simulink model "ssc_Probes_test_all"  (R2019b)
settings: Solver=ode23t  StartTime=0.0  StopTime=10.0  RelTol=1e-3  EnableMultiTasking=on
undefined symbols (not defined in the file): damping_coeff
libraries: fl_lib x88, nesl_utility x71, Pneumatic_lib x16, fl_ps_legacy_lib x1
(part 1 of 4)
settings Model: Creator=tegel  LastModifiedBy=bhisma
settings DataIOCC: LimitDataPoints=on  SaveFormat=Array  ReturnWorkspaceOutputs=off
settings OptimizationCC: ExpressionDepthLimit=2147483647  LifeSpan=inf
settings DebuggingCC: UnderspecifiedInitializationDetection=Classic  MergeDetectMultiDrivingBlocksExec=none  SolverPrmCheckMsg=warning  StateNameClashWarn=warning  SFUnexpectedBacktrackingDiag=warning  SFNoUnconditionalDefaultTransitionDiag=warning  SFExecutionAtInitializationDiag=none  ArithmeticOperatorsInVariantConditions=warning
settings HardwareCC: ProdBitPerPointer=32  ProdBitPerSizeT=32  ProdBitPerPtrDiffT=32  ProdLargestAtomicFloat=None  ProdIntDivRoundTo=Undefined  ProdEndianess=Unspecified  ProdWordSize=32  ProdHWDeviceType=32-bit Generic
settings ModelReferenceCC: PropagateSignalLabelsOutOfModel=off
settings SFSimCC: SimUseLocalCustomCode=off  CustomCodeUndefinedFunction=UseInterfaceOnly
settings RTWCC: RTWUseLocalCustomCode=off
settings CodeAppCC: StateflowObjectComments=on
settings GRTTargetCC: TargetLangStandard=C89/C90 (ANSI)  GeneratePreprocessorConditionals=Disable all
settings ConfigComp: CovMetricSettings=dw  CovHtmlReporting=on  CovSaveCumulativeToWorkspaceVar=on  CovSaveSingleToWorkspaceVar=on  CovExternalEMLEnable=off  CovSFcnEnable=off
settings SimscapeCC: SimscapeNormalizeSystem=off

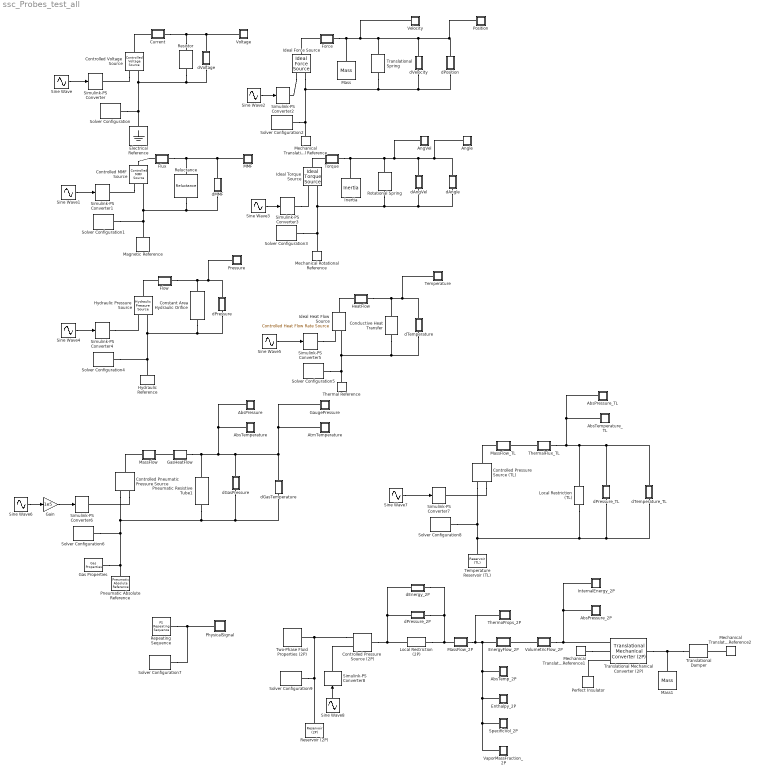
== system ssc_Probes_test_all ==
  AbsPressure : Subsystem  Description=Simscape Probe  InitFcn=|
      | unit=get_param([gcb '/PS-S'],'Unit');                                              
      | set_param(gcb, 'AttributesFormatString', strcat('[', unit,']'));
      mask help: Simscape Probe
      settings: AttributesFormatString=[Pa]
      settings: CopyFcn=|
      | set_param(gcb,'LinkStatus','inactive');
      | set_param(gcb,'LinkStatus','none');
      | set_param([gcb '/Goto'],'GotoTag', [get(gcbh,'name')]);
      | set_param([gcb '/From'],'GotoTag', [get(gcbh,'name')]);
      | h = get_param([gcb, '/PS-S'], 'PortHandles');
      | set(h.Outport(1), 'SignalNameFromLabel', [get(gcbh,'name')])
      | clear h;
      settings: NameChangeFcn=|
      | set_param([gcb '/Goto'],'GotoTag', [get(gcbh,'name')]);
      | set_param([gcb '/From'],'GotoTag', [get(gcbh,'name')]);
      | h = get_param([gcb, '/PS-S'], 'PortHandles');
      | set(h.Outport(1), 'SignalNameFromLabel', [get(gcbh,'name')])
      | clear h;
      settings: OpenFcn=|
      | if exist('logsout', 'var')
      |   vname = get(gcbh,'name');
      |   fHandle = findall(0,'Tag',vname);
      |   if isempty(fHandle)
      |   figure('Tag',vname);
      |   end;
      |   figure(findobj('Tag',vname));
      |   plot(logsout.getElement([gcb, '/PS-S'], '-blockpath').Values)
      |   title(get(gcbh,'name'));
      |   ylabel(['Pressure (' get_param([gcb '/PS-S'],'Unit') ')'] );
      | end
      mask Display: port_label('LConn', 1,'P');
  AbsPressure_2P : Subsystem  Description=Simscape Probe  InitFcn=|
      | unit=get_param([gcb '/PS-S'],'Unit');                                              
      | set_param(gcb, 'AttributesFormatString', strcat('[', unit,']'));
      mask help: Simscape Probe
      settings: AttributesFormatString=[Pa]
      settings: CopyFcn=|
      | set_param(gcb,'LinkStatus','inactive');
      | set_param(gcb,'LinkStatus','none');
      | set_param([gcb '/Goto'],'GotoTag', [get(gcbh,'name')]);
      | set_param([gcb '/From'],'GotoTag', [get(gcbh,'name')]);
      | h = get_param([gcb, '/PS-S'], 'PortHandles');
      | set(h.Outport(1), 'SignalNameFromLabel', [get(gcbh,'name')])
      | clear h;
      settings: NameChangeFcn=|
      | set_param([gcb '/Goto'],'GotoTag', [get(gcbh,'name')]);
      | set_param([gcb '/From'],'GotoTag', [get(gcbh,'name')]);
      | h = get_param([gcb, '/PS-S'], 'PortHandles');
      | set(h.Outport(1), 'SignalNameFromLabel', [get(gcbh,'name')])
      | clear h;
      settings: OpenFcn=|
      | if exist('logsout', 'var')
      |   vname = get(gcbh,'name');
      |   fHandle = findall(0,'Tag',vname);
      |   if isempty(fHandle)
      |   figure('Tag',vname);
      |   end;
      |   figure(findobj('Tag',vname));
      |   plot(logsout.getElement([gcb, '/PS-S'], '-blockpath').Values)
      |   title(get(gcbh,'name'));
      |   ylabel(['Pressure (' get_param([gcb '/PS-S'],'Unit') ')'] );
      | end
      mask Display: port_label('LConn', 1,'P');
  AbsPressure_TL : Subsystem  Description=Simscape Probe  InitFcn=|
      | unit=get_param([gcb '/PS-S'],'Unit');                                              
      | set_param(gcb, 'AttributesFormatString', strcat('[', unit,']'));
      mask help: Simscape Probe
      settings: AttributesFormatString=[Pa]
      settings: CopyFcn=|
      | set_param(gcb,'LinkStatus','inactive');
      | set_param(gcb,'LinkStatus','none');
      | set_param([gcb '/Goto'],'GotoTag', [get(gcbh,'name')]);
      | set_param([gcb '/From'],'GotoTag', [get(gcbh,'name')]);
      | h = get_param([gcb, '/PS-S'], 'PortHandles');
      | set(h.Outport(1), 'SignalNameFromLabel', [get(gcbh,'name')])
      | clear h;
      settings: NameChangeFcn=|
      | set_param([gcb '/Goto'],'GotoTag', [get(gcbh,'name')]);
      | set_param([gcb '/From'],'GotoTag', [get(gcbh,'name')]);
      | h = get_param([gcb, '/PS-S'], 'PortHandles');
      | set(h.Outport(1), 'SignalNameFromLabel', [get(gcbh,'name')])
      | clear h;
      settings: OpenFcn=|
      | if exist('logsout', 'var')
      |   vname = get(gcbh,'name');
      |   fHandle = findall(0,'Tag',vname);
      |   if isempty(fHandle)
      |   figure('Tag',vname);
      |   end;
      |   figure(findobj('Tag',vname));
      |   plot(logsout.getElement([gcb, '/PS-S'], '-blockpath').Values)
      |   title(get(gcbh,'name'));
      |   ylabel(['Pressure (' get_param([gcb '/PS-S'],'Unit') ')'] );
      | end
      mask Display: port_label('LConn', 1,'P');
  AbsTemp_2P : Subsystem  Description=Simscape Probe  InitFcn=|
      | unit=get_param([gcb '/PS-S'],'Unit');                                              
      | set_param(gcb, 'AttributesFormatString', strcat('[', unit,']'));
      mask help: Simscape Probe
      settings: AttributesFormatString=[K]
      settings: CopyFcn=|
      | set_param(gcb,'LinkStatus','inactive');
      | set_param(gcb,'LinkStatus','none');
      | set_param([gcb '/Goto'],'GotoTag', [get(gcbh,'name')]);
      | set_param([gcb '/From'],'GotoTag', [get(gcbh,'name')]);
      | h = get_param([gcb, '/PS-S'], 'PortHandles');
      | set(h.Outport(1), 'SignalNameFromLabel', [get(gcbh,'name')])
      | clear h;
      settings: NameChangeFcn=|
      | set_param([gcb '/Goto'],'GotoTag', [get(gcbh,'name')]);
      | set_param([gcb '/From'],'GotoTag', [get(gcbh,'name')]);
      | h = get_param([gcb, '/PS-S'], 'PortHandles');
      | set(h.Outport(1), 'SignalNameFromLabel', [get(gcbh,'name')])
      | clear h;
      settings: OpenFcn=|
      | if exist('logsout', 'var')
      |   vname = get(gcbh,'name');
      |   fHandle = findall(0,'Tag',vname);
      |   if isempty(fHandle)
      |   figure('Tag',vname);
      |   end;
      |   figure(findobj('Tag',vname));
      |   plot(logsout.getElement([gcb, '/PS-S'], '-blockpath').Values)
      |   title(get(gcbh,'name'));
      |   ylabel(['Temperture (' get_param([gcb '/PS-S'],'Unit') ')'] );
      | end
      mask Display: port_label('LConn', 1,'T');
  AbsTemperature : Subsystem  Description=Simscape Probe  InitFcn=|
      | unit=get_param([gcb '/PS-S'],'Unit');                                              
      | set_param(gcb, 'AttributesFormatString', strcat('[', unit,']'));
      mask help: Simscape Probe
      settings: AttributesFormatString=[K]
      settings: CopyFcn=|
      | set_param(gcb,'LinkStatus','inactive');
      | set_param(gcb,'LinkStatus','none');
      | set_param([gcb '/Goto'],'GotoTag', [get(gcbh,'name')]);
      | set_param([gcb '/From'],'GotoTag', [get(gcbh,'name')]);
      | h = get_param([gcb, '/PS-S'], 'PortHandles');
      | set(h.Outport(1), 'SignalNameFromLabel', [get(gcbh,'name')])
      | clear h;
      settings: NameChangeFcn=|
      | set_param([gcb '/Goto'],'GotoTag', [get(gcbh,'name')]);
      | set_param([gcb '/From'],'GotoTag', [get(gcbh,'name')]);
      | h = get_param([gcb, '/PS-S'], 'PortHandles');
      | set(h.Outport(1), 'SignalNameFromLabel', [get(gcbh,'name')])
      | clear h;
      settings: OpenFcn=|
      | if exist('logsout', 'var')
      |   vname = get(gcbh,'name');
      |   fHandle = findall(0,'Tag',vname);
      |   if isempty(fHandle)
      |   figure('Tag',vname);
      |   end;
      |   figure(findobj('Tag',vname));
      |   plot(logsout.getElement([gcb, '/PS-S'], '-blockpath').Values)
      |   title(get(gcbh,'name'));
      |   ylabel(['Temperature (' get_param([gcb '/PS-S'],'Unit') ')'] );
      | end
      mask Display: port_label('LConn', 1,'T');
  AbsTemperature_TL : Subsystem  Description=Simscape Probe  InitFcn=|
      | unit=get_param([gcb '/PS-S'],'Unit');                                              
      | set_param(gcb, 'AttributesFormatString', strcat('[', unit,']'));
      mask help: Simscape Probe
      settings: AttributesFormatString=[K]
      settings: CopyFcn=|
      | set_param(gcb,'LinkStatus','inactive');
      | set_param(gcb,'LinkStatus','none');
      | set_param([gcb '/Goto'],'GotoTag', [get(gcbh,'name')]);
      | set_param([gcb '/From'],'GotoTag', [get(gcbh,'name')]);
      | h = get_param([gcb, '/PS-S'], 'PortHandles');
      | set(h.Outport(1), 'SignalNameFromLabel', [get(gcbh,'name')])
      | clear h;
      settings: NameChangeFcn=|
      | set_param([gcb '/Goto'],'GotoTag', [get(gcbh,'name')]);
      | set_param([gcb '/From'],'GotoTag', [get(gcbh,'name')]);
      | h = get_param([gcb, '/PS-S'], 'PortHandles');
      | set(h.Outport(1), 'SignalNameFromLabel', [get(gcbh,'name')])
      | clear h;
      settings: OpenFcn=|
      | if exist('logsout', 'var')
      |   vname = get(gcbh,'name');
      |   fHandle = findall(0,'Tag',vname);
      |   if isempty(fHandle)
      |   figure('Tag',vname);
      |   end;
      |   figure(findobj('Tag',vname));
      |   plot(logsout.getElement([gcb, '/PS-S'], '-blockpath').Values)
      |   title(get(gcbh,'name'));
      |   ylabel(['Temperature (' get_param([gcb '/PS-S'],'Unit') ')'] );
      | end
      mask Display: port_label('LConn', 1,'T');
  AngVel : Subsystem  Description=Simscape Probe  InitFcn=|
      | unit=get_param([gcb '/PS-S'],'Unit');                                              
      | set_param(gcb, 'AttributesFormatString', strcat('[', unit,']'));
      mask help: Simscape Probe
      settings: AttributesFormatString=[rad/s]
      settings: CopyFcn=|
      | set_param(gcb,'LinkStatus','inactive');
      | set_param(gcb,'LinkStatus','none');
      | set_param([gcb '/Goto'],'GotoTag', [get(gcbh,'name')]);
      | set_param([gcb '/From'],'GotoTag', [get(gcbh,'name')]);
      | h = get_param([gcb, '/PS-S'], 'PortHandles');
      | set(h.Outport(1), 'SignalNameFromLabel', [get(gcbh,'name')])
      | clear h;
      settings: NameChangeFcn=|
      | set_param([gcb '/Goto'],'GotoTag', [get(gcbh,'name')]);
      | set_param([gcb '/From'],'GotoTag', [get(gcbh,'name')]);
      | h = get_param([gcb, '/PS-S'], 'PortHandles');
      | set(h.Outport(1), 'SignalNameFromLabel', [get(gcbh,'name')])
      | clear h;
      settings: OpenFcn=|
      | if exist('logsout', 'var')
      |   vname = get(gcbh,'name');
      |   fHandle = findall(0,'Tag',vname);
      |   if isempty(fHandle)
      |   figure('Tag',vname);
      |   end;
      |   figure(findobj('Tag',vname));
      |   plot(logsout.getElement([gcb, '/PS-S'], '-blockpath').Values)
      |   title(get(gcbh,'name'));
      |   ylabel(['Anguiar Velocity (' get_param([gcb '/PS-S'],'Unit') ')'] );
      | end
      mask Display: port_label('LConn', 1,'W');
  Angle : Subsystem  Description=Simscape Probe  InitFcn=|
      | unit=get_param([gcb '/PS-S'],'Unit');                                              
      | set_param(gcb, 'AttributesFormatString', strcat('[', unit,']'));
      mask help: Simscape Probe
      settings: AttributesFormatString=[rad]
      settings: CopyFcn=|
      | set_param(gcb,'LinkStatus','inactive');
      | set_param(gcb,'LinkStatus','none');
      | set_param([gcb '/Goto'],'GotoTag', [get(gcbh,'name')]);
      | set_param([gcb '/From'],'GotoTag', [get(gcbh,'name')]);
      | h = get_param([gcb, '/PS-S'], 'PortHandles');
      | set(h.Outport(1), 'SignalNameFromLabel', [get(gcbh,'name')])
      | clear h;
      settings: NameChangeFcn=|
      | set_param([gcb '/Goto'],'GotoTag', [get(gcbh,'name')]);
      | set_param([gcb '/From'],'GotoTag', [get(gcbh,'name')]);
      | h = get_param([gcb, '/PS-S'], 'PortHandles');
      | set(h.Outport(1), 'SignalNameFromLabel', [get(gcbh,'name')])
      | clear h;
      settings: OpenFcn=|
      | if exist('logsout', 'var')
      |   vname = get(gcbh,'name');
      |   fHandle = findall(0,'Tag',vname);
      |   if isempty(fHandle)
      |   figure('Tag',vname);
      |   end;
      |   figure(findobj('Tag',vname));
      |   plot(logsout.getElement([gcb, '/PS-S'], '-blockpath').Values)
      |   title(get(gcbh,'name'));
      |   ylabel(['Angle (' get_param([gcb '/PS-S'],'Unit') ')'] );
      | end
      mask Display: port_label('LConn', 1,'A');
  AtmTemperature : Subsystem  Description=Simscape Probe  InitFcn=|
      | unit=get_param([gcb '/PS-S'],'Unit');                                              
      | set_param(gcb, 'AttributesFormatString', strcat('[', unit,']'));
      mask help: Simscape Probe
      settings: AttributesFormatString=[K]
      settings: CopyFcn=|
      | set_param(gcb,'LinkStatus','inactive');
      | set_param(gcb,'LinkStatus','none');
      | set_param([gcb '/Goto'],'GotoTag', [get(gcbh,'name')]);
      | set_param([gcb '/From'],'GotoTag', [get(gcbh,'name')]);
      | h = get_param([gcb, '/PS-S'], 'PortHandles');
      | set(h.Outport(1), 'SignalNameFromLabel', [get(gcbh,'name')])
      | clear h;
      settings: NameChangeFcn=|
      | set_param([gcb '/Goto'],'GotoTag', [get(gcbh,'name')]);
      | set_param([gcb '/From'],'GotoTag', [get(gcbh,'name')]);
      | h = get_param([gcb, '/PS-S'], 'PortHandles');
      | set(h.Outport(1), 'SignalNameFromLabel', [get(gcbh,'name')])
      | clear h;
      settings: OpenFcn=|
      | if exist('logsout', 'var')
      |   vname = get(gcbh,'name');
      |   fHandle = findall(0,'Tag',vname);
      |   if isempty(fHandle)
      |   figure('Tag',vname);
      |   end;
      |   figure(findobj('Tag',vname));
      |   plot(logsout.getElement([gcb, '/PS-S'], '-blockpath').Values)
      |   title(get(gcbh,'name'));
      |   ylabel(['Temperature (' get_param([gcb '/PS-S'],'Unit') ')'] );
      | end
      mask Display: port_label('LConn', 1,'T');
  Conductive Heat Transfer : fl_lib/Thermal/Thermal Elements/Conductive Heat Transfer  area=1e-4 m^2  thickness=0.1 m  th_cond=401 W/(m*K)  T_specify=off  T_priority=High  T=0 K  T_nominal_specify=off  T_nominal_unit=K  T_nominal_value=1  Q_specify=off  Q_priority=High  Q=0 J/s  Q_nominal_specify=off  Q_nominal_unit=W  Q_nominal_value=1
      settings: SourceProductName=Simscape
  Constant Area Hydraulic Orifice : fl_lib/Hydraulic/Hydraulic Elements/Constant Area Hydraulic Orifice  area=1e-4 m^2  C_d=0.7  lam_spec=2  B_lam=0.999  Re_cr=12  q_specify=off  q_priority=High  q=1 m^3/s  q_nominal_specify=off  q_nominal_unit=m^3/s  q_nominal_value=1  p_specify=off  p_priority=High  p=0 Pa  p_nominal_specify=off  p_nominal_unit=Pa  p_nominal_value=1
      settings: SourceProductName=Simscape  SourceProductBaseCode=SS  InternalSimscapePortConfiguration="{\"Bottom\":[],\"Left\":[{\"id\":\"A\",\"label\":\"A\",\"type\":\"foundation.hydraulic.hydraulic\"}],\"Right\":[{\"id\":\"B\",\"label\":\"B\",\"type\":\"foundation.hydraulic.hydraulic\"}],\"Top\":[]}"
  Controlled MMF Source : fl_lib/Magnetic/Magnetic Sources/Controlled MMF Source
      settings: SourceProductName=Simscape  SourceProductBaseCode=SS  InternalSimscapePortConfiguration="{\"Bottom\":[],\"Left\":[{\"id\":\"N\",\"label\":\"\",\"type\":\"foundation.magnetic.magnetic\"}],\"Right\":[{\"id\":\"mmfI\",\"label\":\"\",\"type\":\"input\"},{\"id\":\"S\",\"label\":\"\",\"type\":\"foundation.magnetic.magnetic\"}],\"Top\":[]}"
  Controlled Pneumatic Pressure Source : Pneumatic_lib/Pneumatic Sources/Controlled Pneumatic Pressure Source
      settings: InternalSimscapePortConfiguration="{\"Bottom\":[],\"Left\":[{\"id\":\"B\",\"label\":\"B\",\"type\":\"foundation.pneumatic.pneumatic\"}],\"Right\":[{\"id\":\"A\",\"label\":\"A\",\"type\":\"foundation.pneumatic.pneumatic\"},{\"id\":\"pressure_difference_reference\",\"label\":\"P\",\"type\":\"input\"}],\"Top\":[]}"
  Controlled Pressure Source (2P) : fl_lib/Two-Phase Fluid/Sources/Controlled Pressure Source (2P)  power_spec=foundation.enum.power_spec.isentropic  area_A=0.01 m^2  area_B=0.01 m^2
      settings: SourceProductName=Simscape  SourceProductBaseCode=SS  InternalSimscapePortConfiguration="{\"Bottom\":[],\"Left\":[{\"id\":\"A\",\"label\":\"A\",\"type\":\"foundation.two_phase_fluid.two_phase_fluid\"},{\"id\":\"P\",\"label\":\"P\",\"type\":\"input\"}],\"Right\":[{\"id\":\"B\",\"label\":\"B\",\"type\":\"foundation.two_phase_fluid.two_phase_fluid\"}],\"Top\":[]}"
  Controlled Pressure Source (TL) : fl_lib/Thermal Liquid/Sources/Controlled Pressure Source (TL)  area=1e-2 m^2
      settings: SourceProductName=Simscape  SourceProductBaseCode=SS  InternalSimscapePortConfiguration="{\"Bottom\":[],\"Left\":[{\"id\":\"A\",\"label\":\"A\",\"type\":\"foundation.thermal_liquid.thermal_liquid\"},{\"id\":\"P\",\"label\":\"P\",\"type\":\"input\"}],\"Right\":[{\"id\":\"B\",\"label\":\"B\",\"type\":\"foundation.thermal_liquid.thermal_liquid\"}],\"Top\":[]}"
  Controlled Voltage Source : fl_lib/Electrical/Electrical Sources/Controlled Voltage Source
  Current : Subsystem  Description=Simscape Probe  InitFcn=|
      | unit=get_param([gcb '/PS-S'],'Unit');                                              
      | set_param(gcb, 'AttributesFormatString', strcat('[', unit,']'));
      mask help: Simscape Probe
      settings: AttributesFormatString=[A]
      settings: CopyFcn=|
      | set_param(gcb,'LinkStatus','inactive');
      | set_param(gcb,'LinkStatus','none');
      | set_param([gcb '/Goto'],'GotoTag', [get(gcbh,'name')]);
      | set_param([gcb '/From'],'GotoTag', [get(gcbh,'name')]);
      | h = get_param([gcb, '/PS-S'], 'PortHandles');
      | set(h.Outport(1), 'SignalNameFromLabel', [get(gcbh,'name')])
      | clear h;
      settings: NameChangeFcn=|
      | set_param([gcb '/Goto'],'GotoTag', [get(gcbh,'name')]);
      | set_param([gcb '/From'],'GotoTag', [get(gcbh,'name')]);
      | h = get_param([gcb, '/PS-S'], 'PortHandles');
      | set(h.Outport(1), 'SignalNameFromLabel', [get(gcbh,'name')])
      | clear h;
      settings: OpenFcn=|
      | if exist('logsout', 'var')
      |   vname = get(gcbh,'name');
      |   fHandle = findall(0,'Tag',vname);
      |   if isempty(fHandle)
      |   figure('Tag',vname);
      |   end;
      |   figure(findobj('Tag',vname));
      |   plot(logsout.getElement([gcb, '/PS-S'], '-blockpath').Values)
      |   title(get(gcbh,'name'));
      |   ylabel(['Current (' get_param([gcb '/PS-S'],'Unit') ')'] );
      | end
      mask Display:
      | patch([0.5 1 0.5], [0.25 .5 0.75],[0.7 0.7 0.7])
      | plot([0,0.5],[0.5,0.5]);
  Electrical Reference : fl_lib/Electrical/Electrical Elements/Electrical Reference
  EnergyFlow_2P : Subsystem  Description=Simscape Probe  InitFcn=|
      | unit=get_param([gcb '/PS-S'],'Unit');                                              
      | set_param(gcb, 'AttributesFormatString', strcat('[', unit,']'));
      mask help: Simscape Probe
      settings: AttributesFormatString=[kW]
      settings: CopyFcn=|
      | if strcmp(get_param(gcb, 'LinkStatus'),'implicit') == 0;
      | set_param(gcb,'LinkStatus','inactive');
      | set_param(gcb,'LinkStatus','none');
      | end
      | set_param([gcb '/Goto'],'GotoTag', [get(gcbh,'name')]);
      | set_param([gcb '/From'],'GotoTag', [get(gcbh,'name')]);
      | h = get_param([gcb, '/PS-S'], 'PortHandles');
      | set(h.Outport(1), 'SignalNameFromLabel', [get(gcbh,'name')])
      | clear h;
      settings: NameChangeFcn=|
      | set_param([gcb '/Goto'],'GotoTag', [get(gcbh,'name')]);
      | set_param([gcb '/From'],'GotoTag', [get(gcbh,'name')]);
      | h = get_param([gcb, '/PS-S'], 'PortHandles');
      | set(h.Outport(1), 'SignalNameFromLabel', [get(gcbh,'name')])
      | clear h;
      settings: OpenFcn=|
      | if exist('logsout', 'var')
      |   vname = get(gcbh,'name');
      |   fHandle = findall(0,'Tag',vname);
      |   if isempty(fHandle)
      |   figure('Tag',vname);
      |   end;
      |   figure(findobj('Tag',vname));
      |   plot(logsout.getElement([gcb, '/PS-S'], '-blockpath').Values)
      |   title(get(gcbh,'name'));
      |   ylabel(['Energy Flow (' get_param([gcb '/PS-S'],'Unit') ')'] );
      | end
      mask Display:
      | patch([0.5 1 0.5], [0.25 .5 0.75],[0.7 0.7 0.7])
      | plot([0,0.5],[0.5,0.5]);
  Enthalpy_2P : Subsystem  Description=Simscape Probe  InitFcn=|
      | unit=get_param([gcb '/PS-S'],'Unit');                                              
      | set_param(gcb, 'AttributesFormatString', strcat('[', unit,']'));
      mask help: Simscape Probe
      settings: AttributesFormatString=[kJ/kg]
      settings: CopyFcn=|
      | set_param(gcb,'LinkStatus','inactive');
      | set_param(gcb,'LinkStatus','none');
      | set_param([gcb '/Goto'],'GotoTag', [get(gcbh,'name')]);
      | set_param([gcb '/From'],'GotoTag', [get(gcbh,'name')]);
      | h = get_param([gcb, '/PS-S'], 'PortHandles');
      | set(h.Outport(1), 'SignalNameFromLabel', [get(gcbh,'name')])
      | clear h;
      settings: NameChangeFcn=|
      | set_param([gcb '/Goto'],'GotoTag', [get(gcbh,'name')]);
      | set_param([gcb '/From'],'GotoTag', [get(gcbh,'name')]);
      | h = get_param([gcb, '/PS-S'], 'PortHandles');
      | set(h.Outport(1), 'SignalNameFromLabel', [get(gcbh,'name')])
      | clear h;
      settings: OpenFcn=|
      | if exist('logsout', 'var')
      |   vname = get(gcbh,'name');
      |   fHandle = findall(0,'Tag',vname);
      |   if isempty(fHandle)
      |   figure('Tag',vname);
      |   end;
      |   figure(findobj('Tag',vname));
      |   plot(logsout.getElement([gcb, '/PS-S'], '-blockpath').Values)
      |   title(get(gcbh,'name'));
      |   ylabel(['Enthalpy (' get_param([gcb '/PS-S'],'Unit') ')'] );
      | end
      mask Display: port_label('LConn', 1,'h');
  Flow : Subsystem  Description=Simscape Probe  InitFcn=|
      | unit=get_param([gcb '/PS-S'],'Unit');                                              
      | set_param(gcb, 'AttributesFormatString', strcat('[', unit,']'));
      mask help: Simscape Probe
      settings: AttributesFormatString=[m^3/s]
      settings: CopyFcn=|
      | set_param(gcb,'LinkStatus','inactive');
      | set_param(gcb,'LinkStatus','none');
      | set_param([gcb '/Goto'],'GotoTag', [get(gcbh,'name')]);
      | set_param([gcb '/From'],'GotoTag', [get(gcbh,'name')]);
      | h = get_param([gcb, '/PS-S'], 'PortHandles');
      | set(h.Outport(1), 'SignalNameFromLabel', [get(gcbh,'name')])
      | clear h;
      settings: NameChangeFcn=|
      | set_param([gcb '/Goto'],'GotoTag', [get(gcbh,'name')]);
      | set_param([gcb '/From'],'GotoTag', [get(gcbh,'name')]);
      | h = get_param([gcb, '/PS-S'], 'PortHandles');
      | set(h.Outport(1), 'SignalNameFromLabel', [get(gcbh,'name')])
      | clear h;
      settings: OpenFcn=|
      | if exist('logsout', 'var')
      |   vname = get(gcbh,'name');
      |   fHandle = findall(0,'Tag',vname);
      |   if isempty(fHandle)
      |   figure('Tag',vname);
      |   end;
      |   figure(findobj('Tag',vname));
      |   plot(logsout.getElement([gcb, '/PS-S'], '-blockpath').Values)
      |   title(get(gcbh,'name'));
      |   ylabel(['Flow (' get_param([gcb '/PS-S'],'Unit') ')'] );
      | end
      mask Display:
      | patch([0.5 1 0.5], [0.25 .5 0.75],[0.7 0.7 0.7])
      | plot([0,0.5],[0.5,0.5]);
  Flux : Subsystem  Description=Simscape Probe  InitFcn=|
      | unit=get_param([gcb '/PS-S'],'Unit');                                              
      | set_param(gcb, 'AttributesFormatString', strcat('[', unit,']'));
      mask help: Simscape Probe
      settings: AttributesFormatString=[Wb]
      settings: CopyFcn=|
      | set_param(gcb,'LinkStatus','inactive');
      | set_param(gcb,'LinkStatus','none');
      | set_param([gcb '/Goto'],'GotoTag', [get(gcbh,'name')]);
      | set_param([gcb '/From'],'GotoTag', [get(gcbh,'name')]);
      | h = get_param([gcb, '/PS-S'], 'PortHandles');
      | set(h.Outport(1), 'SignalNameFromLabel', [get(gcbh,'name')])
      | clear h;
      settings: NameChangeFcn=|
      | set_param([gcb '/Goto'],'GotoTag', [get(gcbh,'name')]);
      | set_param([gcb '/From'],'GotoTag', [get(gcbh,'name')]);
      | h = get_param([gcb, '/PS-S'], 'PortHandles');
      | set(h.Outport(1), 'SignalNameFromLabel', [get(gcbh,'name')])
      | clear h;
      settings: OpenFcn=|
      | if exist('logsout', 'var')
      |   vname = get(gcbh,'name');
      |   fHandle = findall(0,'Tag',vname);
      |   if isempty(fHandle)
      |   figure('Tag',vname);
      |   end;
      |   figure(findobj('Tag',vname));
      |   plot(logsout.getElement([gcb, '/PS-S'], '-blockpath').Values)
      |   title(get(gcbh,'name'));
      |   ylabel(['Flux (' get_param([gcb '/PS-S'],'Unit') ')'] );
      | end
      mask Display:
      | patch([0.5 1 0.5], [0.25 .5 0.75],[0.7 0.7 0.7])
      | plot([0,0.5],[0.5,0.5]);
  Force : Subsystem  Description=Simscape Probe  InitFcn=|
      | unit=get_param([gcb '/PS-S'],'Unit');                                              
      | set_param(gcb, 'AttributesFormatString', strcat('[', unit,']'));
      mask help: Simscape Probe
      settings: AttributesFormatString=[N]
      settings: CopyFcn=|
      | set_param(gcb,'LinkStatus','inactive');
      | set_param(gcb,'LinkStatus','none');
      | set_param([gcb '/Goto'],'GotoTag', [get(gcbh,'name')]);
      | set_param([gcb '/From'],'GotoTag', [get(gcbh,'name')]);
      | h = get_param([gcb, '/PS-S'], 'PortHandles');
      | set(h.Outport(1), 'SignalNameFromLabel', [get(gcbh,'name')])
      | clear h;
      settings: NameChangeFcn=|
      | set_param([gcb '/Goto'],'GotoTag', [get(gcbh,'name')]);
      | set_param([gcb '/From'],'GotoTag', [get(gcbh,'name')]);
      | h = get_param([gcb, '/PS-S'], 'PortHandles');
      | set(h.Outport(1), 'SignalNameFromLabel', [get(gcbh,'name')])
      | clear h;
      settings: OpenFcn=|
      | if exist('logsout', 'var')
      |   vname = get(gcbh,'name');
      |   fHandle = findall(0,'Tag',vname);
      |   if isempty(fHandle)
      |   figure('Tag',vname);
      |   end;
      |   figure(findobj('Tag',vname));
      |   plot(logsout.getElement([gcb, '/PS-S'], '-blockpath').Values)
      |   title(get(gcbh,'name'));
      |   ylabel(['Force (' get_param([gcb '/PS-S'],'Unit') ')'] );
      | end
      mask Display:
      | patch([0.5 1 0.5], [0.25 .5 0.75],[0.7 0.7 0.7])
      | plot([0,0.5],[0.5,0.5]);
  Gain : Gain  Gain=1e5
  Gas Properties : Pneumatic_lib/Pneumatic Utilities/Gas Properties  c_p=1005 J/kg/K  c_v=717.95 J/kg/K  viscosity=18.21e-6 s*Pa  Pa=101325 Pa  Ta=293.15 K  range_error=1
      settings: InternalSimscapePortConfiguration="{\"Bottom\":[],\"Left\":[],\"Right\":[{\"id\":\"A\",\"label\":\"\",\"type\":\"foundation.pneumatic.pneumatic\"}],\"Top\":[]}"
  GasHeatFlow : Subsystem  Description=Simscape Probe  InitFcn=|
      | unit=get_param([gcb '/PS-S'],'Unit');                                              
      | set_param(gcb, 'AttributesFormatString', strcat('[', unit,']'));
      mask help: Simscape Probe
      settings: AttributesFormatString=[J/s]
      settings: CopyFcn=|
      | set_param(gcb,'LinkStatus','inactive');
      | set_param(gcb,'LinkStatus','none');
      | set_param([gcb '/Goto'],'GotoTag', [get(gcbh,'name')]);
      | set_param([gcb '/From'],'GotoTag', [get(gcbh,'name')]);
      | h = get_param([gcb, '/PS-S'], 'PortHandles');
      | set(h.Outport(1), 'SignalNameFromLabel', [get(gcbh,'name')])
      | clear h;
      settings: NameChangeFcn=|
      | set_param([gcb '/Goto'],'GotoTag', [get(gcbh,'name')]);
      | set_param([gcb '/From'],'GotoTag', [get(gcbh,'name')]);
      | h = get_param([gcb, '/PS-S'], 'PortHandles');
      | set(h.Outport(1), 'SignalNameFromLabel', [get(gcbh,'name')])
      | clear h;
      settings: OpenFcn=|
      | if exist('logsout', 'var')
      |   vname = get(gcbh,'name');
      |   fHandle = findall(0,'Tag',vname);
      |   if isempty(fHandle)
      |   figure('Tag',vname);
      |   end;
      |   figure(findobj('Tag',vname));
      |   plot(logsout.getElement([gcb, '/PS-S'], '-blockpath').Values)
      |   title(get(gcbh,'name'));
      |   ylabel(['Heat Flow (' get_param([gcb '/PS-S'],'Unit') ')'] );
      | end
      mask Display:
      | patch([0.5 1 0.5], [0.25 .5 0.75],[0.7 0.7 0.7])
      | plot([0,0.5],[0.5,0.5]);
  GaugePressure : Subsystem  Description=Simscape Probe  InitFcn=|
      | unit=get_param([gcb '/PS-S'],'Unit');                                              
      | set_param(gcb, 'AttributesFormatString', strcat('[', unit,']'));
      mask help: Simscape Probe
      settings: AttributesFormatString=[Pa]
      settings: CopyFcn=|
      | set_param(gcb,'LinkStatus','inactive');
      | set_param(gcb,'LinkStatus','none');
      | set_param([gcb '/Goto'],'GotoTag', [get(gcbh,'name')]);
      | set_param([gcb '/From'],'GotoTag', [get(gcbh,'name')]);
      | h = get_param([gcb, '/PS-S'], 'PortHandles');
      | set(h.Outport(1), 'SignalNameFromLabel', [get(gcbh,'name')])
      | clear h;
      settings: NameChangeFcn=|
      | set_param([gcb '/Goto'],'GotoTag', [get(gcbh,'name')]);
      | set_param([gcb '/From'],'GotoTag', [get(gcbh,'name')]);
      | h = get_param([gcb, '/PS-S'], 'PortHandles');
      | set(h.Outport(1), 'SignalNameFromLabel', [get(gcbh,'name')])
      | clear h;
      settings: OpenFcn=|
      | if exist('logsout', 'var')
      |   vname = get(gcbh,'name');
      |   fHandle = findall(0,'Tag',vname);
      |   if isempty(fHandle)
      |   figure('Tag',vname);
      |   end;
      |   figure(findobj('Tag',vname));
      |   plot(logsout.getElement([gcb, '/PS-S'], '-blockpath').Values)
      |   title(get(gcbh,'name'));
      |   ylabel(['Pressure (' get_param([gcb '/PS-S'],'Unit') ')'] );
      | end
      mask Display: port_label('LConn', 1,'P');
  HeatFlow : Subsystem  Description=Simscape Probe  InitFcn=|
      | unit=get_param([gcb '/PS-S'],'Unit');                                              
      | set_param(gcb, 'AttributesFormatString', strcat('[', unit,']'));
      mask help: Simscape Probe
      settings: AttributesFormatString=[J/s]
      settings: CopyFcn=|
      | set_param(gcb,'LinkStatus','inactive');
      | set_param(gcb,'LinkStatus','none');
      | set_param([gcb '/Goto'],'GotoTag', [get(gcbh,'name')]);
      | set_param([gcb '/From'],'GotoTag', [get(gcbh,'name')]);
      | h = get_param([gcb, '/PS-S'], 'PortHandles');
      | set(h.Outport(1), 'SignalNameFromLabel', [get(gcbh,'name')])
      | clear h;
      settings: NameChangeFcn=|
      | set_param([gcb '/Goto'],'GotoTag', [get(gcbh,'name')]);
      | set_param([gcb '/From'],'GotoTag', [get(gcbh,'name')]);
      | h = get_param([gcb, '/PS-S'], 'PortHandles');
      | set(h.Outport(1), 'SignalNameFromLabel', [get(gcbh,'name')])
      | clear h;
      settings: OpenFcn=|
      | if exist('logsout', 'var')
      |   vname = get(gcbh,'name');
      |   fHandle = findall(0,'Tag',vname);
      |   if isempty(fHandle)
      |   figure('Tag',vname);
      |   end;
      |   figure(findobj('Tag',vname));
      |   plot(logsout.getElement([gcb, '/PS-S'], '-blockpath').Values)
      |   title(get(gcbh,'name'));
      |   ylabel(['Heat Flow (' get_param([gcb '/PS-S'],'Unit') ')'] );
      | end
      mask Display:
      | patch([0.5 1 0.5], [0.25 .5 0.75],[0.7 0.7 0.7])
      | plot([0,0.5],[0.5,0.5]);
  Hydraulic Pressure Source : fl_lib/Hydraulic/Hydraulic Sources/Hydraulic Pressure Source
      settings: SourceProductName=Simscape  SourceProductBaseCode=SS  InternalSimscapePortConfiguration="{\"Bottom\":[],\"Left\":[{\"id\":\"P\",\"label\":\"P\",\"type\":\"foundation.hydraulic.hydraulic\"}],\"Right\":[{\"id\":\"S\",\"label\":\"S\",\"type\":\"input\"},{\"id\":\"T\",\"label\":\"T\",\"type\":\"foundation.hydraulic.hydraulic\"}],\"Top\":[]}"
  Hydraulic Reference : fl_lib/Hydraulic/Hydraulic Elements/Hydraulic Reference
      settings: SourceProductName=Simscape
  Ideal Force Source : fl_lib/Mechanical/Mechanical Sources/Ideal Force Source
  Ideal Heat Flow Source : fl_lib/Thermal/Thermal Sources/Controlled Heat Flow Rate Source
      settings: SourceProductName=Simscape
  Ideal Torque Source : fl_lib/Mechanical/Mechanical Sources/Ideal Torque Source
  Inertia : fl_lib/Mechanical/Rotational Elements/Inertia  inertia=0.01 kg*m^2  w_specify=on  w_priority=High  w=0 rad/s  w_nominal_specify=off  w_nominal_unit=rad/s  w_nominal_value=1  t_specify=off  t_priority=High  t=0 N*m  t_nominal_specify=off  t_nominal_unit=N*m  t_nominal_value=1
  InternalEnergy_2P : Subsystem  Description=Simscape Probe  InitFcn=|
      | unit=get_param([gcb '/PS-S'],'Unit');                                              
      | set_param(gcb, 'AttributesFormatString', strcat('[', unit,']'));
      mask help: Simscape Probe
      settings: AttributesFormatString=[kJ/kg]
      settings: CopyFcn=|
      | set_param(gcb,'LinkStatus','inactive');
      | set_param(gcb,'LinkStatus','none');
      | set_param([gcb '/Goto'],'GotoTag', [get(gcbh,'name')]);
      | set_param([gcb '/From'],'GotoTag', [get(gcbh,'name')]);
      | h = get_param([gcb, '/PS-S'], 'PortHandles');
      | set(h.Outport(1), 'SignalNameFromLabel', [get(gcbh,'name')])
      | clear h;
      settings: NameChangeFcn=|
      | set_param([gcb '/Goto'],'GotoTag', [get(gcbh,'name')]);
      | set_param([gcb '/From'],'GotoTag', [get(gcbh,'name')]);
      | h = get_param([gcb, '/PS-S'], 'PortHandles');
      | set(h.Outport(1), 'SignalNameFromLabel', [get(gcbh,'name')])
      | clear h;
      settings: OpenFcn=|
      | if exist('logsout', 'var')
      |   vname = get(gcbh,'name');
      |   fHandle = findall(0,'Tag',vname);
      |   if isempty(fHandle)
      |   figure('Tag',vname);
      |   end;
      |   figure(findobj('Tag',vname));
      |   plot(logsout.getElement([gcb, '/PS-S'], '-blockpath').Values)
      |   title(get(gcbh,'name'));
      |   ylabel(['Internal Energy (' get_param([gcb '/PS-S'],'Unit') ')'] );
      | end
      mask Display: port_label('LConn', 1,'U');
  Local Restriction (2P) : fl_lib/Two-Phase Fluid/Elements/Local Restriction (2P)  restriction_area=0.001 m^2  area=0.01 m^2  Cd=0.7  B_lam=0.999
      settings: SourceProductName=Simscape  SourceProductBaseCode=SS  InternalSimscapePortConfiguration="{\"Bottom\":[],\"Left\":[{\"id\":\"A\",\"label\":\"A\",\"type\":\"foundation.two_phase_fluid.two_phase_fluid\"}],\"Right\":[{\"id\":\"B\",\"label\":\"B\",\"type\":\"foundation.two_phase_fluid.two_phase_fluid\"}],\"Top\":[]}"
  Local Restriction (TL) : fl_lib/Thermal Liquid/Elements/Local Restriction (TL)  restriction_type=foundation.enum.restriction_type.fixed  restriction_area=1e-5 m^2  min_area=1e-10 m^2  max_area=0.005 m^2  area=1e-2 m^2  Cd=0.7  pressure_recovery=0  Re_c=12
      settings: SourceProductName=Simscape  SourceProductBaseCode=SS
  MMF : Subsystem  Description=Simscape Probe  InitFcn=|
      | unit=get_param([gcb '/PS-S'],'Unit');                                              
      | set_param(gcb, 'AttributesFormatString', strcat('[', unit,']'));
      mask help: Simscape Probe
      settings: AttributesFormatString=[A]
      settings: CopyFcn=|
      | set_param(gcb,'LinkStatus','inactive');
      | set_param(gcb,'LinkStatus','none');
      | set_param([gcb '/Goto'],'GotoTag', [get(gcbh,'name')]);
      | set_param([gcb '/From'],'GotoTag', [get(gcbh,'name')]);
      | h = get_param([gcb, '/PS-S'], 'PortHandles');
      | set(h.Outport(1), 'SignalNameFromLabel', [get(gcbh,'name')])
      | clear h;
      settings: NameChangeFcn=|
      | set_param([gcb '/Goto'],'GotoTag', [get(gcbh,'name')]);
      | set_param([gcb '/From'],'GotoTag', [get(gcbh,'name')]);
      | h = get_param([gcb, '/PS-S'], 'PortHandles');
      | set(h.Outport(1), 'SignalNameFromLabel', [get(gcbh,'name')])
      | clear h;
      settings: OpenFcn=|
      | if exist('logsout', 'var')
      |   vname = get(gcbh,'name');
      |   fHandle = findall(0,'Tag',vname);
      |   if isempty(fHandle)
      |   figure('Tag',vname);
      |   end;
      |   figure(findobj('Tag',vname));
      |   plot(logsout.getElement([gcb, '/PS-S'], '-blockpath').Values)
      |   title(get(gcbh,'name'));
      |   ylabel(['MMF (' get_param([gcb '/PS-S'],'Unit') ')'] );
      | end
      mask Display: port_label('LConn', 1,'F');
  Magnetic Reference : fl_lib/Magnetic/Magnetic Elements/Magnetic Reference
      settings: SourceProductName=Simscape  SourceProductBaseCode=SS  InternalSimscapePortConfiguration="{\"Bottom\":[],\"Left\":[{\"id\":\"M\",\"label\":\"\",\"type\":\"foundation.magnetic.magnetic\"}],\"Right\":[],\"Top\":[]}"
  Mass : fl_lib/Mechanical/Translational Elements/Mass  mass=1 kg  v_specify=on  v_priority=High  v=0 m/s  v_nominal_specify=off  v_nominal_unit=m/s  v_nominal_value=1  f_specify=off  f_priority=High  f=0 N  f_nominal_specify=off  f_nominal_unit=N  f_nominal_value=1
  Mass1 : fl_lib/Mechanical/Translational Elements/Mass  mass=mass kg  v_specify=off  v_priority=High  v=0 m/s  v_nominal_specify=off  v_nominal_unit=m/s  v_nominal_value=1  f_specify=off  f_priority=None  f=0 N  f_nominal_specify=off  f_nominal_unit=N  f_nominal_value=1
  MassFlow : Subsystem  Description=Simscape Probe  InitFcn=|
      | unit=get_param([gcb '/PS-S'],'Unit');                                              
      | set_param(gcb, 'AttributesFormatString', strcat('[', unit,']'));
      mask help: Simscape Probe
      settings: AttributesFormatString=[kg/s]
      settings: CopyFcn=|
      | set_param(gcb,'LinkStatus','inactive');
      | set_param(gcb,'LinkStatus','none');
      | set_param([gcb '/Goto'],'GotoTag', [get(gcbh,'name')]);
      | set_param([gcb '/From'],'GotoTag', [get(gcbh,'name')]);
      | h = get_param([gcb, '/PS-S'], 'PortHandles');
      | set(h.Outport(1), 'SignalNameFromLabel', [get(gcbh,'name')])
      | clear h;
      settings: NameChangeFcn=|
      | set_param([gcb '/Goto'],'GotoTag', [get(gcbh,'name')]);
      | set_param([gcb '/From'],'GotoTag', [get(gcbh,'name')]);
      | h = get_param([gcb, '/PS-S'], 'PortHandles');
      | set(h.Outport(1), 'SignalNameFromLabel', [get(gcbh,'name')])
      | clear h;
      settings: OpenFcn=|
      | if exist('logsout', 'var')
      |   vname = get(gcbh,'name');
      |   fHandle = findall(0,'Tag',vname);
      |   if isempty(fHandle)
      |   figure('Tag',vname);
      |   end;
      |   figure(findobj('Tag',vname));
      |   plot(logsout.getElement([gcb, '/PS-S'], '-blockpath').Values)
      |   title(get(gcbh,'name'));
      |   ylabel(['Mass Flow (' get_param([gcb '/PS-S'],'Unit') ')'] );
      | end
      mask Display:
      | patch([0.5 1 0.5], [0.25 .5 0.75],[0.7 0.7 0.7])
      | plot([0,0.5],[0.5,0.5]);
  MassFlow_2P : Subsystem  Description=Simscape Probe  InitFcn=|
      | unit=get_param([gcb '/PS-S'],'Unit');                                              
      | set_param(gcb, 'AttributesFormatString', strcat('[', unit,']'));
      mask help: Simscape Probe
      settings: AttributesFormatString=[kg/s]
      settings: CopyFcn=|
      | if strcmp(get_param(gcb, 'LinkStatus'),'implicit') == 0;
      | set_param(gcb,'LinkStatus','inactive');
      | set_param(gcb,'LinkStatus','none');
      | end
      | set_param([gcb '/Goto'],'GotoTag', [get(gcbh,'name')]);
      | set_param([gcb '/From'],'GotoTag', [get(gcbh,'name')]);
      | h = get_param([gcb, '/PS-S'], 'PortHandles');
      | set(h.Outport(1), 'SignalNameFromLabel', [get(gcbh,'name')])
      | clear h;
      settings: NameChangeFcn=|
      | set_param([gcb '/Goto'],'GotoTag', [get(gcbh,'name')]);
      | set_param([gcb '/From'],'GotoTag', [get(gcbh,'name')]);
      | h = get_param([gcb, '/PS-S'], 'PortHandles');
      | set(h.Outport(1), 'SignalNameFromLabel', [get(gcbh,'name')])
      | clear h;
      settings: OpenFcn=|
      | if exist('logsout', 'var')
      |   vname = get(gcbh,'name');
      |   fHandle = findall(0,'Tag',vname);
      |   if isempty(fHandle)
      |   figure('Tag',vname);
      |   end;
      |   figure(findobj('Tag',vname));
      |   plot(logsout.getElement([gcb, '/PS-S'], '-blockpath').Values)
      |   title(get(gcbh,'name'));
      |   ylabel(['Mass Flow (' get_param([gcb '/PS-S'],'Unit') ')'] );
      | end
      mask Display:
      | patch([0.5 1 0.5], [0.25 .5 0.75],[0.7 0.7 0.7])
      | plot([0,0.5],[0.5,0.5]);
  MassFlow_TL : Subsystem  Description=Simscape Probe  InitFcn=|
      | unit=get_param([gcb '/PS-S'],'Unit');                                              
      | set_param(gcb, 'AttributesFormatString', strcat('[', unit,']'));
      mask help: Simscape Probe
      settings: AttributesFormatString=[kg/s]
      settings: CopyFcn=|
      | set_param(gcb,'LinkStatus','inactive');
      | set_param(gcb,'LinkStatus','none');
      | set_param([gcb '/Goto'],'GotoTag', [get(gcbh,'name')]);
      | set_param([gcb '/From'],'GotoTag', [get(gcbh,'name')]);
      | h = get_param([gcb, '/PS-S'], 'PortHandles');
      | set(h.Outport(1), 'SignalNameFromLabel', [get(gcbh,'name')])
      | clear h;
      settings: NameChangeFcn=|
      | set_param([gcb '/Goto'],'GotoTag', [get(gcbh,'name')]);
      | set_param([gcb '/From'],'GotoTag', [get(gcbh,'name')]);
      | h = get_param([gcb, '/PS-S'], 'PortHandles');
      | set(h.Outport(1), 'SignalNameFromLabel', [get(gcbh,'name')])
      | clear h;
      settings: OpenFcn=|
      | if exist('logsout', 'var')
      |   vname = get(gcbh,'name');
      |   fHandle = findall(0,'Tag',vname);
      |   if isempty(fHandle)
      |   figure('Tag',vname);
      |   end;
      |   figure(findobj('Tag',vname));
      |   plot(logsout.getElement([gcb, '/PS-S'], '-blockpath').Values)
      |   title(get(gcbh,'name'));
      |   ylabel(['Mass Flow (' get_param([gcb '/PS-S'],'Unit') ')'] );
      | end
      mask Display:
      | patch([0.5 1 0.5], [0.25 .5 0.75],[0.7 0.7 0.7])
      | plot([0,0.5],[0.5,0.5]);
  Mechanical Translational Reference1 : fl_lib/Mechanical/Translational Elements/Mechanical Translational Reference
  Mechanical Translational Reference2 : fl_lib/Mechanical/Translational Elements/Mechanical Translational Reference
  Mechanical Rotational Reference : fl_lib/Mechanical/Rotational Elements/Mechanical Rotational Reference
  Mechanical Translational Reference : fl_lib/Mechanical/Translational Elements/Mechanical Translational Reference
  Perfect Insulator : fl_lib/Thermal/Thermal Elements/Perfect Insulator  T_specify=off  T_priority=None  T=0 K  T_nominal_specify=off  T_nominal_unit=K  T_nominal_value=1
      settings: SourceProductName=Simscape
  PhysicalSignal : Subsystem  Description=Simscape Probe  InitFcn=|
      | unit=get_param([gcb '/PS-S'],'Unit');                                              
      | set_param(gcb, 'AttributesFormatString', strcat('[', unit,']'));
      mask help: Simscape Probe
      settings: AttributesFormatString=[1]
      settings: CopyFcn=|
      | set_param(gcb,'LinkStatus','inactive');
      | set_param(gcb,'LinkStatus','none');
      | set_param([gcb '/Goto'],'GotoTag', [get(gcbh,'name')]);
      | set_param([gcb '/From'],'GotoTag', [get(gcbh,'name')]);
      | h = get_param([gcb, '/PS-S'], 'PortHandles');
      | set(h.Outport(1), 'SignalNameFromLabel', [get(gcbh,'name')])
      | clear h;
      settings: NameChangeFcn=|
      | set_param([gcb '/Goto'],'GotoTag', [get(gcbh,'name')]);
      | set_param([gcb '/From'],'GotoTag', [get(gcbh,'name')]);
      | h = get_param([gcb, '/PS-S'], 'PortHandles');
      | set(h.Outport(1), 'SignalNameFromLabel', [get(gcbh,'name')])
      | clear h;
      settings: OpenFcn=|
      | if exist('logsout', 'var')
      |   vname = get(gcbh,'name');
      |   fHandle = findall(0,'Tag',vname);
      |   if isempty(fHandle)
      |   figure('Tag',vname);
      |   end;
      |   figure(findobj('Tag',vname));
      |   plot(logsout.getElement([gcb, '/PS-S'], '-blockpath').Values)
      |   title(get(gcbh,'name'));
      |   ylabel(['Physical Signal (' get_param([gcb '/PS-S'],'Unit') ')'] );
      | end
      mask Display: disp('PS');
  Pneumatic Absolute Reference : Pneumatic_lib/Pneumatic Elements/Pneumatic Absolute Reference
      settings: InternalSimscapePortConfiguration="{\"Bottom\":[],\"Left\":[{\"id\":\"A\",\"label\":\"\",\"type\":\"foundation.pneumatic.pneumatic\"}],\"Right\":[],\"Top\":[]}"
  Pneumatic Resistive Tube1 : Pneumatic_lib/Pneumatic Elements/Pneumatic Resistive Tube  Diameter=0.01 m  Length=10 m  EquivalentLength=0 m  Roughness=1.5e-5 m  Re_lam=2000  Re_turb=4000  G_specify=off  G_priority=None  G=0 kg/s  G_nominal_specify=off  G_nominal_unit=kg/s  G_nominal_value=1  Q1_specify=off  Q1_priority=None  Q1=0 J/s  Q1_nominal_specify=off  Q1_nominal_unit=J/s  Q1_nominal_value=1  Q2_specify=off  Q2_priority=None  Q2=0 J/s  Q2_nominal_specify=off  Q2_nominal_unit=J/s  Q2_nominal_value=1  p1_specify=off  p1_priority=None  p1=1e+5 Pa  p1_nominal_specify=off  p1_nominal_unit=Pa  p1_nominal_value=1  p2_specify=off  p2_priority=None  p2=1e+5 Pa  p2_nominal_specify=off  p2_nominal_unit=Pa  p2_nominal_value=1  T1_specify=off  T1_priority=None  T1=300 K  T1_nominal_specify=off  T1_nominal_unit=K  T1_nominal_value=1  T2_specify=off  T2_priority=None  T2=300 K  T2_nominal_specify=off  T2_nominal_unit=K  T2_nominal_value=1
      settings: InternalSimscapePortConfiguration="{\"Bottom\":[],\"Left\":[{\"id\":\"A\",\"label\":\"A\",\"type\":\"foundation.pneumatic.pneumatic\"}],\"Right\":[{\"id\":\"B\",\"label\":\"B\",\"type\":\"foundation.pneumatic.pneumatic\"}],\"Top\":[]}"
  Position : Subsystem  Description=Simscape Probe  InitFcn=|
      | unit=get_param([gcb '/PS-S'],'Unit');                                              
      | set_param(gcb, 'AttributesFormatString', strcat('[', unit,']'));
      mask help: Simscape Probe
      settings: AttributesFormatString=[m]
      settings: CopyFcn=|
      | set_param(gcb,'LinkStatus','inactive');
      | set_param(gcb,'LinkStatus','none');
      | set_param([gcb '/Goto'],'GotoTag', [get(gcbh,'name')]);
      | set_param([gcb '/From'],'GotoTag', [get(gcbh,'name')]);
      | h = get_param([gcb, '/PS-S'], 'PortHandles');
      | set(h.Outport(1), 'SignalNameFromLabel', [get(gcbh,'name')])
      | clear h;
      settings: NameChangeFcn=|
      | set_param([gcb '/Goto'],'GotoTag', [get(gcbh,'name')]);
      | set_param([gcb '/From'],'GotoTag', [get(gcbh,'name')]);
      | h = get_param([gcb, '/PS-S'], 'PortHandles');
      | set(h.Outport(1), 'SignalNameFromLabel', [get(gcbh,'name')])
      | clear h;
      settings: OpenFcn=|
      | if exist('logsout', 'var')
      |   vname = get(gcbh,'name');
      |   fHandle = findall(0,'Tag',vname);
      |   if isempty(fHandle)
      |   figure('Tag',vname);
      |   end;
      |   figure(findobj('Tag',vname));
      |   plot(logsout.getElement([gcb, '/PS-S'], '-blockpath').Values)
      |   title(get(gcbh,'name'));
      |   ylabel(['Position (' get_param([gcb '/PS-S'],'Unit') ')'] );
      | end
      mask Display: port_label('LConn', 1,'P');
  Pressure : Subsystem  Description=Simscape Probe  InitFcn=|
      | unit=get_param([gcb '/PS-S'],'Unit');                                              
      | set_param(gcb, 'AttributesFormatString', strcat('[', unit,']'));
      mask help: Simscape Probe
      settings: AttributesFormatString=[Pa]
      settings: CopyFcn=|
      | set_param(gcb,'LinkStatus','inactive');
      | set_param(gcb,'LinkStatus','none');
      | set_param([gcb '/Goto'],'GotoTag', [get(gcbh,'name')]);
      | set_param([gcb '/From'],'GotoTag', [get(gcbh,'name')]);
      | h = get_param([gcb, '/PS-S'], 'PortHandles');
      | set(h.Outport(1), 'SignalNameFromLabel', [get(gcbh,'name')])
      | clear h;
      settings: NameChangeFcn=|
      | set_param([gcb '/Goto'],'GotoTag', [get(gcbh,'name')]);
      | set_param([gcb '/From'],'GotoTag', [get(gcbh,'name')]);
      | h = get_param([gcb, '/PS-S'], 'PortHandles');
      | set(h.Outport(1), 'SignalNameFromLabel', [get(gcbh,'name')])
      | clear h;
      settings: OpenFcn=|
      | if exist('logsout', 'var')
      |   vname = get(gcbh,'name');
      |   fHandle = findall(0,'Tag',vname);
      |   if isempty(fHandle)
      |   figure('Tag',vname);
      |   end;
      |   figure(findobj('Tag',vname));
      |   plot(logsout.getElement([gcb, '/PS-S'], '-blockpath').Values)
      |   title(get(gcbh,'name'));
      |   ylabel(['Pressure (' get_param([gcb '/PS-S'],'Unit') ')'] );
      | end
      mask Display: port_label('LConn', 1,'P');
  Reluctance : fl_lib/Magnetic/Magnetic Elements/Reluctance  g=0.001 m  CSA=0.01 m^2  mur=1  phi_specify=off  phi_priority=High  phi=0 Wb  phi_nominal_specify=off  phi_nominal_unit=Wb  phi_nominal_value=1  mmf_specify=off  mmf_priority=High  mmf=0 A  mmf_nominal_specify=off  mmf_nominal_unit=A  mmf_nominal_value=1
      settings: SourceProductName=Simscape  SourceProductBaseCode=SS  InternalSimscapePortConfiguration="{\"Bottom\":[],\"Left\":[{\"id\":\"N\",\"label\":\"N\",\"type\":\"foundation.magnetic.magnetic\"}],\"Right\":[{\"id\":\"S\",\"label\":\"S\",\"type\":\"foundation.magnetic.magnetic\"}],\"Top\":[]}"
  Repeating Sequence : fl_lib/Physical Signals/Sources/PS Repeating Sequence  y_init=0  offset=0 s  sig_type=1  durations=[ 1 1 ] s  y_start=[ 0 2 ]  y_end=[ 1 1 ]
      settings: SourceProductName=Simscape  SourceProductBaseCode=SS  InternalSimscapePortConfiguration="{\"Bottom\":[],\"Left\":[],\"Right\":[{\"id\":\"Y\",\"label\":\"Y\",\"type\":\"output\"}],\"Top\":[]}"
  Reservoir (2P) : fl_lib/Two-Phase Fluid/Elements/Reservoir (2P)  pressure_spec=2  reservoir_pressure=p0 MPa  energy_spec=foundation.enum.energy_spec.temperature  reservoir_temperature=T0 K  reservoir_quality=0.2  reservoir_void_fraction=0.5  reservoir_enthalpy=1500 kJ/kg  reservoir_internal_energy=1500 kJ/kg  area_A=0.01 m^2
      settings: SourceProductName=Simscape  SourceProductBaseCode=SS
  Resistor : fl_lib/Electrical/Electrical Elements/Resistor  R=1 Ohm  i_specify=off  i_priority=High  i=0 A  i_nominal_specify=off  i_nominal_unit=A  i_nominal_value=1  v_specify=off  v_priority=High  v=0 V  v_nominal_specify=off  v_nominal_unit=V  v_nominal_value=1
  Rotational Spring : fl_lib/Mechanical/Rotational Elements/Rotational Spring  spr_rate=10 N*m/rad  w_specify=off  w_priority=High  w=0 rad/s  w_nominal_specify=off  w_nominal_unit=rad/s  w_nominal_value=1  t_specify=off  t_priority=High  t=0 N*m  t_nominal_specify=off  t_nominal_unit=N*m  t_nominal_value=1  phi_specify=on  phi_priority=High  phi=0 rad  phi_nominal_specify=off  phi_nominal_unit=rad  phi_nominal_value=1
      settings: SourceProductName=Simscape
  Simulink-PS Converter8 : nesl_utility/Simulink-PS Converter  PhysicalDomain=network_engine_domain  SubClassName=ps_input  LeftPortType=input  RightPortType=output  PseudoPeriodic=off  Frequencies=[]  NoiseDistribution=none  NoiseParameters=[]  Unit=MPa  AffineConversion=off  FilteringAndDerivatives=zero  SimscapeFilterOrder=1  InputFilterTimeConstant=0.001  UdotUserProvided=1
  Simulink-PS Converter{,1..5,7} (7 alike) : nesl_utility/Simulink-PS Converter  PhysicalDomain=network_engine_domain  SubClassName=ps_input  LeftPortType=input  RightPortType=output  PseudoPeriodic=off  Frequencies=[]  NoiseDistribution=none  NoiseParameters=[]  Unit=1  AffineConversion=off  FilteringAndDerivatives=zero  SimscapeFilterOrder=1  InputFilterTimeConstant=.001  UdotUserProvided=[]
  Simulink-PS Converter6 : nesl_utility/Simulink-PS Converter  PhysicalDomain=network_engine_domain  SubClassName=ps_input  LeftPortType=input  RightPortType=output  PseudoPeriodic=off  Frequencies=[]  NoiseDistribution=none  NoiseParameters=[]  Unit=1  AffineConversion=off  FilteringAndDerivatives=zero  SimscapeFilterOrder=1  InputFilterTimeConstant=.001  UdotUserProvided=1
  Sine Wave{,1..5,7} (7 alike) : Sin  SampleTime=0
  Sine Wave6 : Sin  Bias=10  SampleTime=0
  Sine Wave8 : Sin  Amplitude=0.0100  SampleTime=0
  Solver Configuration9 : nesl_utility/Solver Configuration  PhysicalDomain=network_engine_domain  SubClassName=solver  LeftPortType=input  RightPortType=generic  Tones=[]  Harmonics=[]  SimulateNoise=off  Profile=off  UseLocalSampling=off  EnableSwitchedLinearOptims=on  FrequencyDomain=off  UseCCode=off  RelTol=0.001  AbsTol=1e-06  MinStep=1e-09  ToWorkspace=off  RevertToSquareIcSolve=off  NumHomotopyIterations=100  PhasorMode=off  PhasorModeNumHarmonics=1  DoDC=off  ResidualTolerance=1e-9  UseLocalSolver=off  LocalSolverChoice=NE_BACKWARD_EULER_ADVANCER  LocalSolverSampleTime=0.001  DoFixedCost=off  MaxNonlinIter=3  MaxModeIter=2  LinearAlgebra=Sparse  EquationFormulation=NE_TIME_EF  DelaysMemoryBudget=1024  AutomaticFiltering=on  FilteringTimeConstant=0.001  PartitionStorageMethod=AS_NEEDED  PartitionMemoryBudget=1024  PartitionMethod=FAST
  Solver Configuration{,1..8} (9 alike) : nesl_utility/Solver Configuration  PhysicalDomain=network_engine_domain  SubClassName=solver  LeftPortType=input  RightPortType=generic  Tones=[]  Harmonics=[]  SimulateNoise=off  Profile=off  UseLocalSampling=off  EnableSwitchedLinearOptims=on  FrequencyDomain=off  UseCCode=off  RelTol=0.001  AbsTol=1e-06  MinStep=1e-09  ToWorkspace=off  RevertToSquareIcSolve=off  NumHomotopyIterations=100  PhasorMode=off  PhasorModeNumHarmonics=1  DoDC=off  ResidualTolerance=1e-9  UseLocalSolver=off  LocalSolverChoice=NE_BACKWARD_EULER_ADVANCER  LocalSolverSampleTime=.001  DoFixedCost=off  MaxNonlinIter=3  MaxModeIter=2  LinearAlgebra=Sparse  EquationFormulation=NE_TIME_EF  DelaysMemoryBudget=1024  AutomaticFiltering=on  FilteringTimeConstant=0.001  PartitionStorageMethod=AS_NEEDED  PartitionMemoryBudget=1024  PartitionMethod=FAST
  SpecificVol_2P : Subsystem  Description=Simscape Probe  InitFcn=|
      | unit=get_param([gcb '/PS-S'],'Unit');                                              
      | set_param(gcb, 'AttributesFormatString', strcat('[', unit,']'));
      mask help: Simscape Probe
      settings: AttributesFormatString=[m^3/kg]
      settings: CopyFcn=|
      | set_param(gcb,'LinkStatus','inactive');
      | set_param(gcb,'LinkStatus','none');
      | set_param([gcb '/Goto'],'GotoTag', [get(gcbh,'name')]);
      | set_param([gcb '/From'],'GotoTag', [get(gcbh,'name')]);
      | h = get_param([gcb, '/PS-S'], 'PortHandles');
      | set(h.Outport(1), 'SignalNameFromLabel', [get(gcbh,'name')])
      | clear h;
      settings: NameChangeFcn=|
      | set_param([gcb '/Goto'],'GotoTag', [get(gcbh,'name')]);
      | set_param([gcb '/From'],'GotoTag', [get(gcbh,'name')]);
      | h = get_param([gcb, '/PS-S'], 'PortHandles');
      | set(h.Outport(1), 'SignalNameFromLabel', [get(gcbh,'name')])
      | clear h;
      settings: OpenFcn=|
      | if exist('logsout', 'var')
      |   vname = get(gcbh,'name');
      |   fHandle = findall(0,'Tag',vname);
      |   if isempty(fHandle)
      |   figure('Tag',vname);
      |   end;
      |   figure(findobj('Tag',vname));
      |   plot(logsout.getElement([gcb, '/PS-S'], '-blockpath').Values)
      |   title(get(gcbh,'name'));
      |   ylabel(['Specific Volume (' get_param([gcb '/PS-S'],'Unit') ')'] );
      | end
      mask Display: port_label('LConn', 1,'V');
  Temperature : Subsystem  Description=Simscape Probe  InitFcn=|
      | unit=get_param([gcb '/PS-S'],'Unit');                                              
      | set_param(gcb, 'AttributesFormatString', strcat('[', unit,']'));
      mask help: Simscape Probe
      settings: AttributesFormatString=[K]
      settings: CopyFcn=|
      | set_param(gcb,'LinkStatus','inactive');
      | set_param(gcb,'LinkStatus','none');
      | set_param([gcb '/Goto'],'GotoTag', [get(gcbh,'name')]);
      | set_param([gcb '/From'],'GotoTag', [get(gcbh,'name')]);
      | h = get_param([gcb, '/PS-S'], 'PortHandles');
      | set(h.Outport(1), 'SignalNameFromLabel', [get(gcbh,'name')])
      | clear h;
      settings: NameChangeFcn=|
      | set_param([gcb '/Goto'],'GotoTag', [get(gcbh,'name')]);
      | set_param([gcb '/From'],'GotoTag', [get(gcbh,'name')]);
      | h = get_param([gcb, '/PS-S'], 'PortHandles');
      | set(h.Outport(1), 'SignalNameFromLabel', [get(gcbh,'name')])
      | clear h;
      settings: OpenFcn=|
      | if exist('logsout', 'var')
      |   vname = get(gcbh,'name');
      |   fHandle = findall(0,'Tag',vname);
      |   if isempty(fHandle)
      |   figure('Tag',vname);
      |   end;
      |   figure(findobj('Tag',vname));
      |   plot(logsout.getElement([gcb, '/PS-S'], '-blockpath').Values)
      |   title(get(gcbh,'name'));
      |   ylabel(['Temperature (' get_param([gcb '/PS-S'],'Unit') ')'] );
      | end
      mask Display: port_label('LConn', 1,'T');
  Temperature Reservoir (TL) : fl_lib/Thermal Liquid/Elements/Reservoir (TL)  pressure_spec=1  reservoir_pressure=0.101325 MPa  reservoir_temperature=293.15 K  area=1e-2 m^2
      settings: SourceProductName=Simscape  SourceProductBaseCode=SS
  Thermal Reference : fl_lib/Thermal/Thermal Elements/Thermal Reference
  ThermalFlux_TL : Subsystem  Description=Simscape Probe  InitFcn=|
      | unit=get_param([gcb '/PS-S'],'Unit');                                              
      | set_param(gcb, 'AttributesFormatString', strcat('[', unit,']'));
      mask help: Simscape Probe
      settings: AttributesFormatString=[J/s]
      settings: CopyFcn=|
      | set_param(gcb,'LinkStatus','inactive');
      | set_param(gcb,'LinkStatus','none');
      | set_param([gcb '/Goto'],'GotoTag', [get(gcbh,'name')]);
      | set_param([gcb '/From'],'GotoTag', [get(gcbh,'name')]);
      | h = get_param([gcb, '/PS-S'], 'PortHandles');
      | set(h.Outport(1), 'SignalNameFromLabel', [get(gcbh,'name')])
      | clear h;
      settings: NameChangeFcn=|
      | set_param([gcb '/Goto'],'GotoTag', [get(gcbh,'name')]);
      | set_param([gcb '/From'],'GotoTag', [get(gcbh,'name')]);
      | h = get_param([gcb, '/PS-S'], 'PortHandles');
      | set(h.Outport(1), 'SignalNameFromLabel', [get(gcbh,'name')])
      | clear h;
      settings: OpenFcn=|
      | if exist('logsout', 'var')
      |   vname = get(gcbh,'name');
      |   fHandle = findall(0,'Tag',vname);
      |   if isempty(fHandle)
      |   figure('Tag',vname);
      |   end;
      |   figure(findobj('Tag',vname));
      |   plot(logsout.getElement([gcb, '/PS-S'], '-blockpath').Values)
      |   title(get(gcbh,'name'));
      |   ylabel(['Thermal Flux (' get_param([gcb '/PS-S'],'Unit') ')'] );
      | end
      mask Display:
      | patch([0.5 1 0.5], [0.25 .5 0.75],[0.7 0.7 0.7])
      | plot([0,0.5],[0.5,0.5]);
  ThermoProps_2P : Subsystem  Description=Simscape Probe  InitFcn=|
      | %unit=get_param([gcb '/PS-S'],'Unit');                                              
      | %set_param(gcb, 'AttributesFormatString', strcat('[', unit,']'));
      mask help: Simscape Probe
      settings: CopyFcn=|
      | if strcmp(get_param(gcb, 'LinkStatus'),'implicit') == 0;
      | set_param(gcb,'LinkStatus','inactive');
      | set_param(gcb,'LinkStatus','none');
      | end
      | set_param([gcb '/Goto'],'GotoTag', [get(gcbh,'name')]);
      | set_param([gcb '/From'],'GotoTag', [get(gcbh,'name')]);
      | h = get_param([gcb, '/PS-S'], 'PortHandles');
      | set(h.Outport(1), 'SignalNameFromLabel', [get(gcbh,'name')])
      | clear h;
      settings: NameChangeFcn=|
      | set_param([gcb '/Goto'],'GotoTag', [get(gcbh,'name')]);
      | set_param([gcb '/From'],'GotoTag', [get(gcbh,'name')]);
      | %h = get_param([gcb, '/PS-S'], 'PortHandles');
      | %set(h.Outport(1), 'SignalNameFromLabel', [get(gcbh,'name')])
      | %clear h;
      settings: OpenFcn=|
      | if exist('logsout', 'var')
      |   vname = get(gcbh,'name');
      |   fHandle = findall(0,'Tag',vname);
      |   if isempty(fHandle)
      |   figure('Tag',vname);
      |   end;
      |   figure(findobj('Tag',vname));
      |   subplot(2,2,1);
      |   plot(logsout.getElement([gcb, '/PS-S1'], '-blockpath').Values);
      |   title('Absolute Temperature','Interpreter','none');
      |   ylabel(['Temperature (' get_param([gcb '/PS-S1'],'Unit') ')'] );
      |   subplot(2,2,2);
      |   plot(logsout.getElement([gcb, '/PS-S2'], '-blockpath').Values);
      |   title('Enthalpy','Interpreter','none');
      |   ylabel(['Enthalpy (' get_param([gcb '/PS-S2'],'Unit') ')'] );
      |   subplot(2,2,3);
      |   plot(logsout.getElement([gcb, '/PS-S3'], '-blockpath').Values);
      |   title('Specific Volume','Interpreter','none');
      |   ylabel(['Volume (' get_param([gcb '/PS-S3'],'Unit') ')'] );
      |   subplot(2,2,4);
      |   plot(logsout.getElement([gcb, '/PS-S4'], '-blockpath').Values);
      |   title('Vapor Mass Fraction','Interpreter','none');
      |   ylabel('Mass Fraction (-)')
      | end
      mask Display: port_label('LConn', 1,'TP');
  Torque : Subsystem  Description=Simscape Probe  InitFcn=|
      | unit=get_param([gcb '/PS-S'],'Unit');                                              
      | set_param(gcb, 'AttributesFormatString', strcat('[', unit,']'));
      mask help: Simscape Probe
      settings: AttributesFormatString=[N*m]
      settings: CopyFcn=|
      | set_param(gcb,'LinkStatus','inactive');
      | set_param(gcb,'LinkStatus','none');
      | set_param([gcb '/Goto'],'GotoTag', [get(gcbh,'name')]);
      | set_param([gcb '/From'],'GotoTag', [get(gcbh,'name')]);
      | h = get_param([gcb, '/PS-S'], 'PortHandles');
      | set(h.Outport(1), 'SignalNameFromLabel', [get(gcbh,'name')])
      | clear h;
      settings: NameChangeFcn=|
      | set_param([gcb '/Goto'],'GotoTag', [get(gcbh,'name')]);
      | set_param([gcb '/From'],'GotoTag', [get(gcbh,'name')]);
      | h = get_param([gcb, '/PS-S'], 'PortHandles');
      | set(h.Outport(1), 'SignalNameFromLabel', [get(gcbh,'name')])
      | clear h;
      settings: OpenFcn=|
      | if exist('logsout', 'var')
      |   vname = get(gcbh,'name');
      |   fHandle = findall(0,'Tag',vname);
      |   if isempty(fHandle)
      |   figure('Tag',vname);
      |   end;
      |   figure(findobj('Tag',vname));
      |   plot(logsout.getElement([gcb, '/PS-S'], '-blockpath').Values)
      |   title(get(gcbh,'name'));
      |   ylabel(['Torque (' get_param([gcb '/PS-S'],'Unit') ')'] );
      | end
      mask Display:
      | patch([0.5 1 0.5], [0.25 .5 0.75],[0.7 0.7 0.7])
      | plot([0,0.5],[0.5,0.5]);
  Translational Spring : fl_lib/Mechanical/Translational Elements/Translational Spring  spr_rate=1000 N/m  v_specify=off  v_priority=High  v=0 m/s  v_nominal_specify=off  v_nominal_unit=m/s  v_nominal_value=1  f_specify=off  f_priority=High  f=0 N  f_nominal_specify=off  f_nominal_unit=N  f_nominal_value=1  x_specify=on  x_priority=High  x=0 m  x_nominal_specify=off  x_nominal_unit=m  x_nominal_value=1
  Translational Mechanical Converter (2P) : fl_lib/Two-Phase Fluid/Elements/Translational Mechanical Converter (2P)  mech_orientation=1  interface_area=0.01 m^2  length_init=0 m  dead_volume=1e-3 m^3  area_A=0.01 m^2  pressure_spec=2  environment_pressure=0.101325 MPa  energy_spec=foundation.enum.energy_spec.temperature  p_init=p0 MPa  T_init=T0 K  x_init=0.2  alpha_init=0.5  h_init=1500 kJ/kg  u_init=1500 kJ/kg  time_constant=0.1 s
      settings: SourceProductName=Simscape  SourceProductBaseCode=SS  InternalSimscapePortConfiguration="{\"Bottom\":[],\"Left\":[{\"id\":\"A\",\"label\":\"A\",\"type\":\"foundation.two_phase_fluid.two_phase_fluid\"},{\"id\":\"C\",\"label\":\"C\",\"type\":\"foundation.mechanical.translational.translational\"},{\"id\":\"H\",\"label\":\"H\",\"type\":\"foundation.thermal.thermal\"}],\"Right\":[{\"id\":\"R\",\"label\":\"R\",\"type\":\"foundation.mechanical.translational.translational\"}],\"Top\":[]}"
  Translational Damper : fl_lib/Mechanical/Translational Elements/Translational Damper  D=damping_coeff N/(m/s)  v_specify=off  v_priority=None  v=0 m/s  v_nominal_specify=off  v_nominal_unit=m/s  v_nominal_value=1  f_specify=off  f_priority=None  f=0 N  f_nominal_specify=off  f_nominal_unit=N  f_nominal_value=1
  Two-Phase Fluid Properties (2P) : fl_lib/Two-Phase Fluid/Utilities/Two-Phase Fluid Properties (2P)  u_min=30 kJ/kg  u_max=4000 kJ/kg  unorm_liq=[- 1; - 0.958333333333333; - 0.916666666666667; - 0.875000000000000; - 0.833333333333333; - 0.791666666666667; - 0.750000000000000; - 0.708333333333333; - 0.666666666666667; - 0.625000000000000; - 0.583333333333333; - 0.541666666666667; - 0.500000000000000; - 0.458333333333333; - 0.416666666666667; - 0.375000000000000; - 0.333333333333333; - 0.291666666666667; - 0.250000000000000; - 0.208333333333333; - 0.166666666666667; - 0.125000000000000; - 0.0833333333333334; - 0.0416666666666666; 0]  unorm_vap=[1; 1.04166666666667; 1.08333333333333; 1.12500000000000; 1.16666666666667; 1.20833333333333; 1.25000000000000; 1.29166666666667; 1.33333333333333; 1.37500000000000; 1.41666666666667; 1.45833333333333; 1.50000000000000; 1.54166666666667; 1.58333333333333; 1.62500000000000; 1.66666666666667; 1.70833333333333; 1.75000000000000; 1.79166666666667; 1.83333333333333; 1.87500000000000; 1.91666666666667; 1.95833333333333; 2]  p_TLU=[0.0100000000000000; 0.0113196254062952; 0.0128133919338844; 0.0145042796875616; 0.0164183012851334; 0.0185849020355406; 0.0210374129255013; 0.0238135633834228; 0.0269560617089414; 0.0305132520974195; 0.0345398583670641; 0.0390978258301657; 0.0442572742598049; 0.0500975766124663; 0.0567085801016295; 0.0641919884073333; 0.0726629262856258; 0.0822517106478526; 0.0931058553560676; 0.105392340576339; 0.119300181601685; 0.135043336663406; 0.152863998464597; 0.173036320072773; 0.195870632490759; 0.221718218788951; 0.250976718244193; 0.284096243622557; 0.321586305714293; 0.364023651648013; 0.412061137568721; 0.466437772176980; 0.527990085639029; 0.597664998767154; 0.676534390449808; 0.765811587436809; 0.866870030158498; 0.981264401733804; 1.11075454521590; 1.25733253701838; 1.42325333301949; 1.61106945880418; 1.82367027771861; 2.06432644083690; 2.33674020265844; 2.64510237659239; 2.99415680643271; 3.38927334565274; 3.83653046723300; 4.34280877489164; 4.91589685429451; 5.56461109265990; 6.29893131006251; 7.13015428898921; 8.07106756404470; 9.13614614538857; 10.3417752022967; 11.7065021326111; 13.2513218959154; 15.0000000000000] MPa  v_liq=[0.00100014653127097, 0.00100014589056495, 0.00100014516531303, 0.00100014434435927, 0.00100014341507570, 0.00100014236316846, 0.00100014117245773, 0.00100013982462919, 0.00100013829895221, 0.00100013657196175, 0.00100013461709724, 0.00100013240429428, 0.00100012989952355, 0.00100012706426724, 0.00100012385492768, 0.00100012022215802, 0.00100011611010459, 0.00100011145554972, 0.00100010618694160, 0.00100010022329700, 0.00100009347295965, 0.00100008583219596, 0.00100007718360550, 0.00100006739432461, 0.00100005631399353, 0.00100004377245774, 0.00100002957717009, 0.00100001351025157, 0.000999995325171353, 0.000999974742993171, 0.000999951448135311, 0.000999925083575715, 0.000999895245458996, 0.000999861476968741, 0.000999823261448727, 0.000999780014626622, 0.000999731075849002, 0.000999675698203637, 0.000999613037395483, 0.000999542139226026, 0.000999461925512780, 0.000999371178269456, 0.000999268521947446, 0.000999152403527187, 0.000999021070226962, 0.000998872544582274, 0.000998704596635093, 0.000998514712960788, 0.000998300062251834, 0.000998057457181136, 0.000997783312273721, 0.000997473597540044, 0.000997123787664712, 0.000996728806605579, 0.000996282967555572, 0.000995779908341708, 0.000995212522564771, 0.000994572886905826, 0.000993852185535502, 0.000993040632804194; 0.00100024167454484, 0.00100024827446638, 0.00100025506729129, 0.00100026205360356, 0.00100026923314535, 0.00100027660466718, 0.00100028416575324, 0.00100029191263605, 0.00100029983996455, 0.00100030794055453, 0.00100031620509806, 0.00100032462183378, 0.00100033317617063, 0.00100034185026028, 0.00100035062251038, 0.00100035946703093, 0.00100036835300528, 0.00100037724397555, 0.00100038609703205, 0.00100039486189162, 0.00100040347985407, 0.00100041188261830, 0.00100041999093887, 0.00100042771310849, 0.00100043494323437, 0.00100044155929159, 0.00100044742091892, 0.00100045236692768, 0.00100045621248618, 0.00100045874593946, 0.00100045972522020, 0.00100045887379963, 0.00100045587612270, 0.00100045037246646, 0.00100044195315304, 0.00100043015204231, 0.00100041443922155, 0.00100039421277810, 0.00100036878970630, 0.00100033739548888, 0.00100029915270092, 0.00100025306821598, 0.00100019801886911, 0.00100013273593363, 0.00100005578746814, 0.000999965559342127, 0.000999860234323345, 0.000999737769470378, 0.000999595871914015, 0.000999431973327368, 0.000999243203655958, 0.000999026365133722, 0.000998777908373732, 0.000998493913645907, 0.000998170082832452, 0.000997801752063760, 0.000997383944315996, 0.000996911503116873, 0.000996379412562607, 0.000995783649594471; 0.00100037271474781, 0.00100039112951782, 0.00100041036465722, 0.00100043044734279, 0.00100045140527759, 0.00100047326663115, 0.00100049605995216, 0.00100051981410388, 0.00100054455812924, 0.00100057032113023, 0.00100059713211033, 0.00100062501978846, 0.00100065401238112, 0.00100068413734578, 0.00100071542108122, 0.00100074788857851, 0.00100078156301498, 0.00100081646528391, 0.00100085261345040, 0.00100089002212421, 0.00100092870173695, 0.00100096865771195, 0.00100100988951019, 0.00100105238954661, 0.00100109614192926, 0.00100114112104921, 0.00100118728995098, 0.00100123459848678, 0.00100128298121757, 0.00100133235503079, 0.00100138261644146, 0.00100143363853832, 0.00100148526753519, 0.00100153731888219, 0.00100158957288937, 0.00100164176981209, 0.00100169360434481, 0.00100174471946743, 0.00100179469959108, 0.00100184306294895, 0.00100188925318864, 0.00100193263012947, 0.00100197245967270, 0.00100200790297952, 0.00100203800445688, 0.00100206167990502, 0.00100207770362353, 0.00100208469595409, 0.00100208111163530, 0.00100206523025012, 0.00100203515073722, 0.00100198879318191, 0.00100192391315890, 0.00100183813768971, 0.00100172903824909, 0.00100159426929360, 0.00100143182689682, 0.00100124054504200, 0.00100102113320357, 0.00100077876343579; 0.00100053820502829, 0.00100057273009268, 0.00100060901514394, 0.00100064712536559, 0.00100068712835574, 0.00100072909418559, 0.00100077309542693, 0.00100081920724885, ...(+27551 chars)] m^3/kg  v_vap=[14.6701298526143, 13.0555604501595, 11.6192850042735, 10.3415439624948, 9.20477465163709, 8.19336634148034, 7.29344317494033, 6.49266980885039, 5.78008078222277, 5.14592754302288, 4.58154303464320, 4.07922134962491, 3.63211080345366, 3.23411893861451, 2.87982812198215, 2.56442055203874, 2.28361162425560, 2.03359072072320, 1.81096859468511, 1.61273061346637, 1.43619520570816, 1.27897693200308, 1.13895366300397, 1.01423740677890, 0.903148378421264, 0.804191950425798, 0.716038162749803, 0.637503507367755, 0.567534734000954, 0.505194452013786, 0.449648328610578, 0.400153705796730, 0.356049478397011, 0.316747093031554, 0.281722543581877, 0.250509252555236, 0.222691740070170, 0.197899993113076, 0.175804457409188, 0.156111582849460, 0.138559861039561, 0.122916300297237, 0.108973289415702, 0.0965458068190992, 0.0854689364381787, 0.0755956557967383, 0.0667948654692325, 0.0589496322607289, 0.0519556211509164, 0.0457196932017009, 0.0401586482294805, 0.0351980920150038, 0.0307714078679363, 0.0268188106985457, 0.0232864567074083, 0.0201255697686738, 0.0172915176288723, 0.0147427020157611, 0.0124389359490747, 0.0103383641950851; 16.7705069537463, 14.9051638146331, 13.2479324681934, 11.7755197027496, 10.4672469731054, 9.30475616119939, 8.27174849103437, 7.35375297468595, 6.53792083909057, 5.81284320473033, 5.16838927787860, 4.59556277218081, 4.08637449996837, 3.63372930784914, 3.23132573848935, 2.87356698305257, 2.55548185099455, 2.27265462773203, 2.02116281824523, 1.79752188779567, 1.59863621126872, 1.42175553164247, 1.26443630702150, 1.12450739570081, 1.00003959084572, 0.889318571491166, 0.790820885462615, 0.703192623211907, 0.625230480057784, 0.555864938480502, 0.494145332423895, 0.439226582440883, 0.390357414359384, 0.346869895284528, 0.308170139488956, 0.273730053343684, 0.243080003144836, 0.215802302709297, 0.191525429134439, 0.169918885313967, 0.150688636824553, 0.133573065814166, 0.118339351714924, 0.104780292910687, 0.0927114530704765, 0.0819686355506332, 0.0724056345715589, 0.0638922330175475, 0.0563124178758865, 0.0495627868398671, 0.0435511211966039, 0.0381950993957258, 0.0334211360523469, 0.0291633026997556, 0.0253623229772657, 0.0219645834382973, 0.0189210911095282, 0.0161862262022392, 0.0137159311336892, 0.0114643029795147; 18.8601950215919, 16.7457844069409, 14.8690703751678, 13.2032553530326, 11.7245717987526, 10.4119362359156, 9.24664734837487, 8.21211571839204, 7.29362472334359, 6.47811863234659, 5.75401470408389, 5.11103657535340, 4.54006657153218, 4.03301472510086, 3.58270263966173, 3.18276050830723, 2.82753579348204, 2.51201224513943, 2.23173808433543, 1.98276231264539, 1.76157822586876, 1.56507331514428, 1.39048483135679, 1.23536037093818, 1.09752291404566, 0.975039810710567, 0.866195304782806, 0.769465988528140, 0.683499338074383, 0.607094381000494, 0.539184676097011, 0.478823186318730, 0.425168855815559, 0.377474698769303, 0.335077229576392, 0.297387083232355, 0.263880691872724, 0.234092898557282, 0.207610402772849, 0.184065943973894, 0.163133139957595, 0.144521906138152, 0.127974389980195, 0.113261362090582, 0.100179011861433, 0.0885461012256339, 0.0782014351527822, 0.0690016107194192, 0.0608190209018881, 0.0535400555344017, 0.0470635171312157, 0.0412991788264867, 0.0361664824105577, 0.0315933528135328, 0.0275150696960877, 0.0238731792293544, 0.0206143447160611, 0.0176889801890720, 0.0150492788370285, 0.0126455386898903; 20.9225998352962, 18.5625301819548, 16.4693335718467, 14.6127563267345, 12.9659821422015, 11.5052407729468, 10.2094613143216, 9.05996509679292, 8.04019347955838, 7.13546674210594, 6.33277042383440, 5.62056600735728, 4.98862316609506, 4.42787111525588, 3.93026688745328, 3.48867860274118, 3.09678202330668, 2.74896887826064, 2.44026561684563, 2.16626140150730, 1.92304428790128, 1.70714465904389, 1.51548508723124, 1.34533589162175, 1.19427574288739, 1.06015674032681, 0.941073452380807, 0.835335469567849, 0.741443070311525, 0.658065645721636, 0.584022569779633, 0.518266237158298, 0.459867022601904, ...(+24054 chars)] m^3/kg  s_liq=[0.108418558232296, 0.108418558207709, 0.108418558176574, 0.108418558136355, 0.108418558085427, 0.108418558019576, 0.108418557935229, 0.108418557827078, 0.108418557688324, 0.108418557511082, 0.108418557284235, 0.108418556991943, 0.108418556618412, 0.108418556139622, 0.108418555526093, 0.108418554739449, 0.108418553737724, 0.108418552458695, 0.108418550812083, 0.108418548700198, 0.108418545994407, 0.108418542527900, 0.108418538086078, 0.108418532395616, 0.108418525108764, 0.108418515780799, 0.108418503846267, 0.108418488583248, 0.108418469069983, 0.108418444127046, 0.108418412247908, 0.108418370066307, 0.108418317135978, 0.108418249327477, 0.108418162463102, 0.108418051191365, 0.108417908657720, 0.108417726088220, 0.108417492246682, 0.108417192749588, 0.108416809186707, 0.108416317993932, 0.108415689016181, 0.108414883672517, 0.108413852609806, 0.108412532707491, 0.108410843259770, 0.108408681104004, 0.108405914414838, 0.108402374805481, 0.108397847273680, 0.108392057412871, 0.108384655182220, 0.108375194312792, 0.108363106225798, 0.108347665760105, 0.108327954346015, 0.108302801103478, 0.108270720901750, 0.108229831438241; 0.132402075233730, 0.133913152967641, 0.135450632491540, 0.137015295314324, 0.138607953364168, 0.140229450960470, 0.141880665967836, 0.143562513835149, 0.145275948156807, 0.147021963917748, 0.148801600028085, 0.150615942110757, 0.152466125491614, 0.154353338395260, 0.156278825352761, 0.158243890854529, 0.160249903261465, 0.162298298999423, 0.164390587075258, 0.166528353917508, 0.168713268633122, 0.170947088685541, 0.173231665892747, 0.175568953360890, 0.177961012463284, 0.180410020885331, 0.182918281264376, 0.185488230693510, 0.188122451193997, 0.190823681281565, 0.193594828790127, 0.196438985139926, 0.199359441274861, 0.202359705538252, 0.205443523807925, 0.208614902296096, 0.211878133482685, 0.215237823243126, 0.218698934794862, 0.222266814476769, 0.225947246743319, 0.229746508624330, 0.233671424029330, 0.237729463206844, 0.241928813963973, 0.246278510721084, 0.250788575856960, 0.255470203596043, 0.260335997080883, 0.265400280768215, 0.270679521492925, 0.276192910403818, 0.281963189842230, 0.288017864800513, 0.294391039428519, 0.301126312424400, 0.308281569833382, 0.315937496802269, 0.324214625518394, 0.333315277744489; 0.156249341709312, 0.159253836011265, 0.162309727277652, 0.165418512043650, 0.168581744054898, 0.171801037988994, 0.175078071512166, 0.178414593071916, 0.181812422737190, 0.185273458366014, 0.188799680330327, 0.192393156706225, 0.196056048863478, 0.199790617403185, 0.203599228501172, 0.207484360690495, 0.211448612114120, 0.215494708303773, 0.219625510526078, 0.223844024763324, 0.228153411385118, 0.232556995600529, 0.237058278647489, 0.241660950646219, 0.246368902786307, 0.251186243048528, 0.256117311554463, 0.261166698166682, 0.266339261731557, 0.271640151342055, 0.277074829905523, 0.282649100374995, 0.288369135053695, 0.294241508480465, 0.300273234502147, 0.306471808265626, 0.312845254044419, 0.319402180025039, 0.326151841455526, 0.333104213944177, 0.340270079181024, 0.347661126028397, 0.355290070837777, 0.363170807447191, 0.371318564713365, 0.379750147592603, 0.388484193486860, 0.397541519442633, 0.406945566836472, 0.416722988005763, 0.426904437631796, 0.437525667372150, 0.448629080394090, 0.460266012671596, 0.472500185264831, 0.485413149128963, 0.499113291149146, 0.513751821890250, 0.529554800561924, 0.546901998125236; 0.179961810203108, 0.184442351578967, 0.188997921112655, 0.193630668337565, 0.198342823533958, 0.203136702995362, 0.208014711784644, 0.212979355012542, 0.218033238735088, 0.223179078749959, 0.228419707216622, 0.233758079936863, 0.239197284179369, 0.244740546994841, 0.250391244078285, 0.256152909239680, 0.262029244517986, 0.268024131017151, 0.274141640520313, 0.280386046741590, 0.286761844910038, 0.293273753972341, 0.299926744565099, 0.306726049866520, 0.313677185207314, 0.320785968704364, 0.328058542319842, 0.335501396996210, 0.343121398770024, 0.350925818243373, ...(+23853 chars)] kJ/kg/K  s_vap=[8.14882019342211, 8.10536596221817, 8.06202037227044, 8.01878369080587, 7.97565604079952, 7.93263738307102, 7.88972752099325, 7.84692603021050, 7.80423228135342, 7.76164539287660, 7.71916420402210, 7.67678724225736, 7.63451268658946, 7.59233832721822, 7.55026152112611, 7.50827914349165, 7.46638753481084, 7.42458244365619, 7.38285896504682, 7.34121147443834, 7.29963355735276, 7.25811793464848, 7.21665638335877, 7.17523965289152, 7.13385737615743, 7.09249797486916, 7.05114855780039, 7.00979481020818, 6.96842087187959, 6.92700920036901, 6.88554041493573, 6.84399311547874, 6.80234366939930, 6.76056595780591, 6.71863107079645, 6.67650693968241, 6.63415789188560, 6.59154411171677, 6.54862098712041, 6.50533831841537, 6.46163935957201, 6.41745965489722, 6.37272562300410, 6.32735282389364, 6.28124382141705, 6.23428551925837, 6.18634580014950, 6.13726922907369, 6.08687147786752, 6.03493196304403, 5.98118391628414, 5.92530066396150, 5.86687617091004, 5.80539667843886, 5.74019803431865, 5.67039894964465, 5.59479125692550, 5.51164717609952, 5.41834873445089, 5.31057516163824; 8.40143902496430, 8.35565822048246, 8.30997919872300, 8.26440226899148, 8.21892761318573, 8.17355527037025, 8.12828511267730, 8.08311683886072, 8.03804993943995, 7.99308367739294, 7.94821705961550, 7.90344880571649, 7.85877731352830, 7.81420062085748, 7.76971636336337, 7.72532172839676, 7.68101340469984, 7.63678752792606, 7.59263962199067, 7.54856453630971, 7.50455637900910, 7.46060844617921, 7.41671314719238, 7.37286192597957, 7.32904517794870, 7.28525216191296, 7.24147090594988, 7.19768810552734, 7.15388901148498, 7.11005730455231, 7.06617495200701, 7.02222204083665, 6.97817658036664, 6.93401426576445, 6.88970819211716, 6.84522850688571, 6.80054198640511, 6.75561151961388, 6.71039547916157, 6.66484695615064, 6.61891282953002, 6.57253273173035, 6.52563743471180, 6.47814742311849, 6.42997068466347, 6.38100014857397, 6.33111042060927, 6.28015361002120, 6.22795391706832, 6.17430048866354, 6.11893778227701, 6.06155216996897, 6.00175323224603, 5.93904586246594, 5.87278880989426, 5.80212948403842, 5.72589672385037, 5.64241237202362, 5.54912894102131, 5.44183510378133; 8.62422353998968, 8.57667696874268, 8.52922420582322, 8.48186554931014, 8.43460136662897, 8.38743167652506, 8.34035643548342, 8.29337544202538, 8.24648830533689, 8.19969442720372, 8.15299297571841, 8.10638285095168, 8.05986265949270, 8.01343067706692, 7.96708480924226, 7.92082254825687, 7.87464092583672, 7.82853646191852, 7.78250510923650, 7.73654219377116, 7.69064235107809, 7.64479945850944, 7.59900656329111, 7.55325580631327, 7.50753834130673, 7.46184424880275, 7.41616252609596, 7.37048069615193, 7.32478509143197, 7.27906049203689, 7.23329004092735, 7.18745508215550, 7.14153497057726, 7.09550684514453, 7.04934535624945, 7.00302233577352, 6.95650639642030, 6.90976244447297, 6.86275108712556, 6.81542791169392, 6.76774260885919, 6.71963790494242, 6.67104825797659, 6.62189825737886, 6.57210064496010, 6.52155384290807, 6.47013882881256, 6.41771509893169, 6.36411563774239, 6.30913969843394, 6.25254385602027, 6.19402897903527, 6.13322185594674, 6.06964880891238, 6.00269501654342, 5.93154155476737, 5.85506129685574, 5.77163591636857, 5.67880366329606, 5.57248753599534; 8.82316936585347, 8.77423364165373, 8.72538380550795, 8.67662024286522, 8.62794323528833, 8.57935294727824, 8.53084940648383, 8.48243249663023, 8.43410192926396, 8.38585722658645, 8.33769769711844, 8.28962240896252, 8.24163016015917, 8.19371944571662, 8.14588842116493, 8.09813486243545, 8.05045612191344, 8.00284908054925, 7.95531009594893, 7.90783494639628, 7.86041877077385, 7.81305600434253, 7.76574031029331, 7.71846450688848, 7.67122048984190, 7.62399914933856, 7.57679028073687, 7.52958248752553, 7.48236307449809, 7.43511792835949, 7.38783138207770, 7.34048605823705, 7.29306268545632, 7.24553988054092, 7.19789388751518, 7.15009826294258, 7.10212349493977, 7.05393654092860, 7.00550026625903, 6.95677276209581, 6.90770651595831, 6.85824740137939, ...(+23003 chars)] kJ/kg/K  T_liq=[280.286790612849, 280.286794818551, 280.286799579421, 280.286804968725, 280.286811069491, 280.286817975611, 280.286825793531, 280.286834643614, 280.286844662283, 280.286856003922, 280.286868843356, 280.286883378485, 280.286899833563, 280.286918462436, 280.286939552630, 280.286963429768, 280.286990463103, 280.287021070522, 280.287055724673, 280.287094962190, 280.287139390949, 280.287189699793, 280.287246669433, 280.287311185120, 280.287384250765, 280.287467005078, 280.287560740277, 280.287666922975, 280.287787218345, 280.287923517733, 280.288077970252, 280.288252923005, 280.288451289791, 280.288676168414, 280.288931151630, 280.289220332616, 280.289548378463, 280.289920615564, 280.290343128493, 280.290822875783, 280.291367824964, 280.291987111104, 280.292691223286, 280.293492224841, 280.294404013838, 280.295442632862, 280.296626638296, 280.297977541918, 280.299520341307, 280.301284158585, 280.303303011893, 280.305616749963, 280.308272187965, 280.311324490948, 280.314838863181, 280.318892527863, 280.323577582756, 280.329003672466, 280.335302067902, 280.342630325621; 281.892229144175, 281.993731863802, 282.097051060458, 282.202241622112, 282.309360634771, 282.418467527855, 282.529624165041, 282.642895131553, 282.758347788427, 282.876052509721, 282.996082873827, 283.118515874278, 283.243432146867, 283.370916213756, 283.501056745300, 283.633946842238, 283.769684339879, 283.908372136457, 284.050118548864, 284.195037697068, 284.343249923927, 284.494882252238, 284.650068873248, 284.808951709655, 284.971680994628, 285.138415938082, 285.309325450262, 285.484588943771, 285.664397224258, 285.848953481746, 286.038474398063, 286.233191388376, 286.433351997307, 286.639221475635, 286.851084567251, 287.069247543611, 287.294040529477, 287.525819999897, 287.764972537493, 288.011917467618, 288.267111646738, 288.531054391516, 288.804292603749, 289.087429258788, 289.381130245052, 289.686135556555, 290.003271775584, 290.333468035274, 290.677776328861, 291.037397870226, 291.413718047531, 291.808353912932, 292.223220509183, 292.660626434777, 293.123416476615, 293.615193361571, 294.140680381075, 294.706358541278, 295.321729982245, 296.002397146969; 283.498772250649, 283.701908099907, 283.908685518010, 284.119214457410, 284.333609262714, 284.551988960103, 284.774477437256, 285.001204016495, 285.232303560631, 285.467916945182, 285.708191438080, 285.953281117399, 286.203347322662, 286.458559137668, 286.719093909399, 286.985137806419, 287.256886419932, 287.534545412943, 287.818331221725, 288.108471815749, 288.405207522545, 288.708791925349, 289.019492833515, 289.337593392757, 289.663393177507, 289.997209560031, 290.339379090793, 290.690259076875, 291.050229322904, 291.419694067818, 291.799084146098, 292.188859408225, 292.589511440835, 293.001566635633, 293.425589665775, 293.862187440075, 294.312013621886, 294.775773818416, 295.254231571517, 295.748215313973, 296.258626498257, 296.786449161908, 297.332761271025, 297.898748669837, 298.485720159636, 299.095129254929, 299.728597919264, 300.387947884548, 301.075240320137, 301.792827422355, 302.543420969011, 303.330185691339, 304.156869892145, 305.027994347154, 305.949134486161, 306.927360303107, 307.971956866715, 309.095692271995, 310.317335271404, 311.667798095961; 285.106293126421, 285.411172602911, 285.721524712785, 286.037514447256, 286.359313374004, 286.687100069935, 287.021060388606, 287.361388318397, 287.708286138491, 288.061965124469, 288.422646114904, 288.790560134461, 289.165949066708, 289.549066374071, 289.940177870867, 290.339562555145, 290.747513503641, 291.164338837901, 291.590362767741, 292.025926635559, 292.471390571288, 292.927133967749, 293.393557791829, 293.871085743315, 294.360166073488, 294.861273530254, 295.374911394926, 295.901613876589, 296.441948655684, 296.996519756975, 297.565970746785, 298.150988311981, 298.752306281096, 299.370710159312, 300.007042263896, 300.662207564799, 301.337180357902, 302.033011927388, 302.750839391823, 303.491895976225, 304.257523017334, 305.049184093832, ...(+23003 chars)] K  T_vap=[318.956328970162, 321.402061570293, 323.891069427645, 326.424584422168, 329.003885925055, 331.630303023024, 334.305215305784, 337.030058254551, 339.806322863648, 342.635559507624, 345.519380515023, 348.459463004775, 351.457551897283, 354.515463057944, 357.635086593879, 360.818390306169, 364.067423303739, 367.384319785044, 370.771302993958, 374.230689356153, 377.764892802165, 381.376429283245, 385.067921485766, 388.842103749247, 392.701827192490, 396.650065050780, 400.689918225727, 404.824621046631, 409.057547239378, 413.392216094575, 417.832298821268, 422.381625065704, 427.044189565786, 431.824158900750, 436.725878281644, 441.753878310480, 446.912881613678, 452.207809227217, 457.643786574641, 463.226148832641, 468.960445418232, 474.852443251931, 480.908128345581, 487.133705121872, 493.535592682155, 500.120416981471, 506.894997518885, 513.866326665861, 521.041539071074, 528.427867600180, 536.032580858680, 543.862895306303, 551.925851969209, 560.228143175488, 568.775867400284, 577.574177852998, 586.626767827288, 595.935091872314, 605.497134571737, 615.305392191820; 363.978536968709, 366.242685213961, 368.544388665973, 370.884603507333, 373.264317734153, 375.684552505962, 378.146362180939, 380.650838231375, 383.199108065769, 385.792337401743, 388.431731394528, 391.118535860856, 393.854038542449, 396.639570389001, 399.476506923322, 402.366269752998, 405.310328321605, 408.310202021310, 411.367462818945, 414.483738579300, 417.660717298846, 420.900152488361, 424.203869959475, 427.573776274581, 431.011869105551, 434.520249711623, 438.101137683530, 441.756888008769, 445.490010387106, 449.303190569200, 453.199313306223, 457.181486293217, 461.253064274111, 465.417672267940, 469.679226691507, 474.041953014626, 478.510398510132, 483.089438669515, 487.784275956398, 492.600429763846, 497.543716708886, 502.620240019060, 507.836302302949, 513.198406783542, 518.713169817069, 524.387253436435, 530.227279164513, 536.239726548909, 542.430813641794, 548.806353849571, 555.371577263717, 562.130884676443, 569.087559111515, 576.243277113506, 583.597513517594, 591.146665346870, 598.882790458991, 606.791669959939, 614.849523609522, 623.016491891088; 409.044376643768, 411.155207313235, 413.299418149787, 415.477760524482, 417.691046184315, 419.940060593800, 422.225628748958, 424.548598961953, 426.909840854914, 429.310246713358, 431.750731551977, 434.232231956414, 436.755707528514, 439.322140397235, 441.932535091576, 444.587918437021, 447.289339558277, 450.037870100202, 452.834604810326, 455.680662660435, 458.577188718118, 461.525357010468, 464.526374647308, 467.581487487319, 470.691987631820, 473.859223014942, 477.084628629879, 480.369672604050, 483.715965518341, 487.125223807634, 490.599304374845, 494.140228214236, 497.750205326212, 501.431660132879, 505.187256407909, 509.019920557817, 512.932861946065, 516.929588845191, 521.013918536779, 525.189980047257, 529.462207987427, 533.835325914609, 538.314317483806, 542.904383279255, 547.610880480633, 552.439241377998, 557.394865387911, 562.482970789425, 567.708446853141, 573.075545285959, 578.587635942998, 584.246745146230, 590.052950155376, 596.003616689153, 602.092175593293, 608.306513055365, 614.626521939866, 621.020248559118, 627.437128419428, 633.794109638232; 453.618577793990, 455.589733567715, 457.591144751017, 459.623439626296, 461.687258501340, 463.783253674947, 465.912088119114, 468.074437529252, 470.270987680865, 472.502434835002, 474.769484877764, 477.072852380790, 479.413259516969, 481.791434796152, 484.208111659168, 486.664026969246, 489.159919465729, 491.696528271543, 494.274591574951, 496.894845637907, 499.558024315083, 502.264859297952, 505.016081323705, 507.812422606552, 510.654620753971, 513.543424420466, 516.479600920166, 519.463945966144, 522.497295623722, 525.580540458896, 528.714641730608, 531.900649321042, 535.139720932557, 538.433141896130, 541.782344765504, 545.188927708868, 548.654670566503, 552.181547325009, 555.771733659420, 559.427608099360, 563.151745252466, 566.946899313424, ...(+23003 chars)] K  nu_liq=[1.42144856213661, 1.42144591084759, 1.42144290971436, 1.42143951258012, 1.42143566719501, 1.42143131442273, 1.42142638731982, 1.42142081012040, 1.42141449705926, 1.42140735106579, 1.42139926226798, 1.42139010630888, 1.42137974243236, 1.42136801133165, 1.42135473270168, 1.42133970247850, 1.42132268969391, 1.42130343297242, 1.42128163654922, 1.42125696567104, 1.42122904153348, 1.42119743549480, 1.42116166253859, 1.42112117387940, 1.42107534861567, 1.42102348429984, 1.42096478627857, 1.42089835567002, 1.42082317579026, 1.42073809683418, 1.42064181860640, 1.42053287517810, 1.42040959891047, 1.42027011426667, 1.42011229906090, 1.41993375575971, 1.41973177646249, 1.41950330362401, 1.41924488608820, 1.41895262990142, 1.41862214342500, 1.41824847619145, 1.41782605095453, 1.41734858838855, 1.41680902393095, 1.41619941627878, 1.41551084718600, 1.41473331234971, 1.41385560336740, 1.41286518111627, 1.41174804133795, 1.41048857383059, 1.40906941746287, 1.40747131435480, 1.40567296800149, 1.40365091564262, 1.40137940319874, 1.39883032385722, 1.39597317541177, 1.39277509886508; 1.35502102531771, 1.35098911183860, 1.34690479176181, 1.34276680565194, 1.33857385355618, 1.33432459187025, 1.33001763251055, 1.32565153467188, 1.32122480586254, 1.31673589608343, 1.31218319406150, 1.30756502302392, 1.30287963616034, 1.29812521178242, 1.29329984818351, 1.28840155813518, 1.28342826300304, 1.27837778644610, 1.27324784763645, 1.26803605400355, 1.26273989333610, 1.25735672524825, 1.25188377229607, 1.24631810933541, 1.24065665329055, 1.23489615096788, 1.22903316612833, 1.22306406526958, 1.21698500198517, 1.21079189975051, 1.20448043292033, 1.19804600569253, 1.19148372878677, 1.18478839349529, 1.17795444274822, 1.17097593872609, 1.16384652650345, 1.15655939843461, 1.14910722702188, 1.14148214135218, 1.13367564786334, 1.12567856048504, 1.11748094003512, 1.10907195387127, 1.10043980779627, 1.09157158059142, 1.08245305953512, 1.07306852446686, 1.06340047122844, 1.05342924772068, 1.04313256207234, 1.03248479876338, 1.02145603848802, 1.01001060769798, 0.998104857129814, 0.985683625461654, 0.972674331113477, 0.958976361686715, 0.944439429788450, 0.928808875789713; 1.29345388679286, 1.28599169627991, 1.27846722241341, 1.27087935694937, 1.26322696976869, 1.25550890591779, 1.24772398705618, 1.23987099972278, 1.23194870073641, 1.22395581044859, 1.21589101008016, 1.20775293860274, 1.19954018941340, 1.19125130695423, 1.18288478321954, 1.17443905413981, 1.16591249585150, 1.15730342080313, 1.14861007370281, 1.13983062727046, 1.13096317776557, 1.12200574024740, 1.11295624377646, 1.10381252486057, 1.09457232397242, 1.08523327695427, 1.07579290934260, 1.06624862865112, 1.05659771614316, 1.04683731771963, 1.03696443379393, 1.02697590796986, 1.01686841433119, 1.00663844308800, 0.996282284279271, 0.985796009177289, 0.975175448922552, 0.964416169814234, 0.953513444524267, 0.942462218273867, 0.931257068723559, 0.919892157912384, 0.908361174011129, 0.896657252138503, 0.884772912172022, 0.872699910635769, 0.860429117308168, 0.847950320953845, 0.835251976281266, 0.822320858840908, 0.809141583883398, 0.795695919444224, 0.781961783070619, 0.767911730080048, 0.753510621148608, 0.738711881911336, 0.723451236311029, 0.707635418167133, 0.691118989275341, 0.673645084345478; 1.23627855183976, 1.22589703534483, 1.21547412533489, 1.20500929029544, 1.19450199980437, 1.18395172155731, 1.17335792453903, 1.16272006433197, 1.15203759196447, 1.14130994632761, 1.13053655232327, 1.11971681856072, 1.10885013495421, 1.09793587042235, 1.08697337064112, 1.07596195583233, 1.06490091861773, 1.05378952188940, 1.04262699671677, 1.03141254243767, 1.02014531361424, 1.00882443975391, 0.997449001208439, 0.986018037775299, 0.974530544173625, 0.962985466547335, 0.951381701080849, 0.939718089095542, 0.927993414106284, 0.916206397398273, 0.904355693125051, 0.892439882628083, 0.880457467809976, 0.868406863361753, 0.856286387592848, 0.844094251552356, 0.831828546050104, 0.819487226083722, 0.807068092016621, ...(+24303 chars)] mm^2/s  nu_vap=[152.226711638926, 136.535839729463, 122.481986619018, 109.892364772812, 98.6126138326657, 88.5048171783214, 79.4457387365774, 71.3252354758992, 64.0448621367446, 57.5166129428771, 51.6618042020237, 46.4100771468747, 41.6985083053968, 37.4708158159140, 33.6766512280004, 30.2709675129326, 27.2134550149750, 24.4680379783231, 22.0024250890197, 19.7877081870173, 17.7980039407342, 16.0101338436589, 14.4033383975240, 12.9590217962026, 11.6605238248981, 10.4929160458454, 9.44281965944515, 8.49824271281678, 7.64843457998392, 6.88375586269470, 6.19556206122107, 5.57609954305216, 5.01841249654781, 4.51625969846393, 4.06404005064608, 3.65672595377926, 3.28980368634688, 2.95922004620898, 2.66133459162473, 2.39287688917938, 2.15090823885904, 1.93278740229482, 1.73613990971805, 1.55883056511999, 1.39893880814850, 1.25473662600421, 1.12466873942344, 1.00733481369779, 0.901473468035447, 0.805947873867884, 0.719732745030166, 0.641902530266420, 0.571620619093685, 0.508129357876729, 0.450740626569377, 0.398826610486498, 0.351810120886297, 0.309153091984898, 0.270339769384995, 0.234843973330048; 200.999093049455, 179.871734279718, 160.985548702038, 144.100700879307, 129.003218806076, 115.502186211829, 103.427240622576, 92.6263468840161, 82.9638102771221, 74.3185083922748, 66.5823148204801, 59.6586944965459, 53.4614518589526, 47.9136150942103, 42.9464415994034, 38.4985314202170, 34.5150368756090, 30.9469578724112, 27.7505135626861, 24.8865820198358, 22.3202005199712, 20.0201198256530, 17.9584065907625, 16.1100886479872, 14.4528385128181, 12.9666909481039, 11.6337908877355, 10.4381684233499, 9.36553791920941, 8.40311864262249, 7.53947458448556, 6.76437140052975, 6.06864863185657, 5.44410556625824, 4.88339928213309, 4.37995357682268, 3.92787762292267, 3.52189332141510, 3.15727043101665, 2.82976865052293, 2.53558591658981, 2.27131249154269, 2.03388913958941, 1.82057104813571, 1.62889462900018, 1.45664824180103, 1.30184593862291, 1.16270395016990, 1.03761959596500, 0.925152321873452, 0.824006573540286, 0.733016163617070, 0.651130123218909, 0.577399146820487, 0.510963025049564, 0.451038042109594, 0.396903568359845, 0.347885799164835, 0.303333643778395, 0.262571844341226; 258.317013220967, 230.714513987028, 206.083600096503, 184.102059075628, 164.482871346891, 146.970267525175, 131.336364308779, 117.378092464578, 104.914477906416, 93.7842244151052, 83.8435613673052, 74.9643276745716, 67.0322674115503, 59.9455117317469, 53.6132275951261, 47.9544147289997, 42.8968344871290, 38.3760560776768, 34.3346072357551, 30.7212178435678, 27.4901462700957, 24.6005793308076, 22.0160977715714, 19.7042000738345, 17.6358781724894, 15.7852393848420, 14.1291707705216, 12.6470340498996, 11.3204045578770, 10.1328284632564, 9.06961095209363, 8.11762649188679, 7.26514963248022, 6.50170411236581, 5.81792828612719, 5.20545510795651, 4.65680510034467, 4.16529090884650, 3.72493219562807, 3.33037975854023, 2.97684788074459, 2.66005402029146, 2.37616504107430, 2.12174926761127, 1.89373371764110, 1.68936593093861, 1.50617987292294, 1.34196539976283, 1.19474120485425, 1.06272984517470, 0.944336158612330, 0.838127010187755, 0.742812908462636, 0.657231249093029, 0.580329805551871, 0.511150860477489, 0.448813999374582, 0.392495176665866, 0.341395520222827, 0.294681076862530; 323.311749912997, 288.293441068685, 257.092138400968, 229.289265240041, 204.512389020052, 182.430111165537, 162.747524159086, 145.202176302921, 129.560480995354, 115.614527277592, 103.179243486901, 92.0898756572568, 82.1997455658483, 73.3782572785791, 65.5091245583267, 58.4887945729971, 52.2250460812127, 46.6357427058629, 41.6477240659304, 37.1958194559230, 33.2219704666858, 29.6744504556659, 26.5071701200861, 23.6790596220649, 21.1535187771674, 18.8979277623819, 16.8832116390446, 15.0834527327927, 13.4755455763389, 12.0388897111200, 10.7551161686205, 9.60784391862870, 8.58246298636039, 7.66594130816766, 6.84665272247479, 6.11422378220823, 5.45939733150859, 4.87391101657608, 4.35038910121004, 3.88224613494465, ...(+23090 chars)] mm^2/s  k_liq=[0.572554404248487, 0.572555310470629, 0.572556336274441, 0.572557497438484, 0.572558811823476, 0.572560299645860, 0.572561983789696, 0.572563890157546, 0.572566048069427, 0.572568490712285, 0.572571255650778, 0.572574385404399, 0.572577928099920, 0.572581938210977, 0.572586477394399, 0.572591615436370, 0.572597431324173, 0.572604014456244, 0.572611466012009, 0.572619900506749, 0.572629447542995, 0.572640253794801, 0.572652485252951, 0.572666329762322, 0.572681999892350, 0.572699736181617, 0.572719810805256, 0.572742531721175, 0.572768247353106, 0.572797351882653, 0.572830291224995, 0.572867569564315, 0.572909757690532, 0.572957500640308, 0.573011527949908, 0.573072664445758, 0.573141842544295, 0.573220116098094, 0.573308675969252, 0.573408867533159, 0.573522210330687, 0.573650420106231, 0.573795433492679, 0.573959435615987, 0.574144890913119, 0.574354577469113, 0.574591625185830, 0.574859558094471, 0.575162341118255, 0.575504431558158, 0.575890835534283, 0.576327169537766, 0.576819727139714, 0.577375550745721, 0.578002508063294, 0.578709372472935, 0.579505907335372, 0.580402950209969, 0.581412497886040, 0.582547787064850; 0.576050800573674, 0.576269203803912, 0.576491191298789, 0.576716874014994, 0.576946368331688, 0.577179796533672, 0.577417287202474, 0.577658976054434, 0.577905006317069, 0.578155529530994, 0.578410706297579, 0.578670707115777, 0.578935713308632, 0.579205918047830, 0.579481527485554, 0.579762762010039, 0.580049857636823, 0.580343067553168, 0.580642663834418, 0.580948939352214, 0.581262209902162, 0.581582816575011, 0.581911128381704, 0.582247545240750, 0.582592501238021, 0.582946468331404, 0.583309960473370, 0.583683538229556, 0.584067813955354, 0.584463457599522, 0.584871203213982, 0.585291856261983, 0.585726301824906, 0.586175513824295, 0.586640565389550, 0.587122640521649, 0.587623047222283, 0.588143231944695, 0.588684797567041, 0.589249520370440, 0.589839372464798, 0.590456545846368, 0.591103478319325, 0.591782887359762, 0.592497802465964, 0.593251607385294, 0.594048086355296, 0.594891478353702, 0.595786540690470, 0.596738624618097, 0.597753766844799, 0.598838802869949, 0.600001511503328, 0.601250805932194, 0.602596997603761, 0.604052180141296, 0.605630824552403, 0.607350784946181, 0.609235246966390, 0.611317443106307; 0.579446354059027, 0.579869496778885, 0.580298728992226, 0.580734218101602, 0.581176138421331, 0.581624671760933, 0.582080007794279, 0.582542345244407, 0.583011892125690, 0.583488866751870, 0.583973498572880, 0.584466029112187, 0.584966712998090, 0.585475819090281, 0.585993631714721, 0.586520452019645, 0.587056599465543, 0.587602413467384, 0.588158255204707, 0.588724509621418, 0.589301587638491, 0.589889928605901, 0.590490003007917, 0.591102315561869, 0.591727408431334, 0.592365865125706, 0.593018314606828, 0.593685435976501, 0.594367963700908, 0.595066693462044, 0.595782488716029, 0.596516288054679, 0.597269113475906, 0.598042079687880, 0.598836404589493, 0.599653421089476, 0.600494590455791, 0.601361517419291, 0.602255967290054, 0.603179885399809, 0.604135419237773, 0.605124943731576, 0.606151090220326, 0.607216780428037, 0.608325262907308, 0.609480160866065, 0.610685523309595, 0.611945888175308, 0.613266357842692, 0.614652691507837, 0.616111420515207, 0.617649995999297, 0.619276983429506, 0.621002328700494, 0.622837736105207, 0.624797232606198, 0.626898059657668, 0.629162201848013, 0.631619380636505, 0.634314362867082; 0.582746367770288, 0.583362505233585, 0.583986413215904, 0.584618288659039, 0.585258335745262, 0.585906766517986, 0.586563801168298, 0.587229669473643, 0.587904610843926, 0.588588875440705, 0.589282725012420, 0.589986433833627, 0.590700289733651, 0.591424595211098, 0.592159668648591, 0.592905845638070, 0.593663480429516, 0.594432947518588, 0.595214643389113, 0.596008988276577, 0.596816429054218, 0.597637440023932, 0.598472527046636, 0.599322229637580, 0.600187124295836, 0.601067828111329, 0.601965002603241, 0.602879358259097, 0.603811659421600, 0.604762729845211, ...(+24509 chars)] W/(m*K)  k_vap=[0.0199421013835313, 0.0201273137338362, 0.0203176574383462, 0.0205133817852906, 0.0207147546971045, 0.0209220643934607, 0.0211356210807621, 0.0213557591612683, 0.0215828391533393, 0.0218172501319896, 0.0220594122682676, 0.0223097796093009, 0.0225688431132828, 0.0228371339593379, 0.0231152212346911, 0.0234037380194701, 0.0237033544118126, 0.0240148019840970, 0.0243388742473494, 0.0246764323057461, 0.0250284110656918, 0.0253958260664840, 0.0257797810109872, 0.0261814760887289, 0.0266022172012042, 0.0270434262207749, 0.0275066524418147, 0.0279935854172907, 0.0285060694182945, 0.0290461198113026, 0.0296159417227084, 0.0302179514586361, 0.0308548012788943, 0.0315294082993457, 0.0322449885341686, 0.0330050974129327, 0.0338136785522496, 0.0346751231788535, 0.0355943434647069, 0.0365768642553124, 0.0376289394149485, 0.0387577015282099, 0.0399713573738314, 0.0412794470335611, 0.0426931926916704, 0.0442259757153838, 0.0458940001475507, 0.0477172318303510, 0.0497207529351877, 0.0519367559576045, 0.0544075458371618, 0.0571901751193038, 0.0603638075738443, 0.0640418037391327, 0.0683923133789705, 0.0736749241479538, 0.0803093387976896, 0.0890124743676502, 0.101095701351753, 0.119191605669304; 0.0234436911363380, 0.0236334162031423, 0.0238277412682283, 0.0240268654112047, 0.0242310016712489, 0.0244403782984729, 0.0246552400100384, 0.0248758496943685, 0.0251024898304280, 0.0253354643538189, 0.0255751005870464, 0.0258217513623452, 0.0260757973519435, 0.0263376496260020, 0.0266077524684126, 0.0268865864843032, 0.0271746720396929, 0.0274725730811168, 0.0277808994800796, 0.0281003188500550, 0.0284315519927676, 0.0287753850922845, 0.0291326750174147, 0.0295043569667193, 0.0298914531211196, 0.0302950824471601, 0.0307164718103406, 0.0311569685764842, 0.0316180549010163, 0.0321013639338159, 0.0326086982043373, 0.0331420505033467, 0.0337036276512690, 0.0342958776493391, 0.0349215208628172, 0.0355835861051872, 0.0362854528053454, 0.0370309008832956, 0.0378241705852531, 0.0386700354094380, 0.0395738924950263, 0.0405418779651975, 0.0415810096837861, 0.0426993817511930, 0.0439064154201657, 0.0452132001385198, 0.0466329599996708, 0.0481817033593695, 0.0498791439301748, 0.0517500324524313, 0.0538261240575849, 0.0561491575642728, 0.0587754964132257, 0.0617836021852648, 0.0652865389480323, 0.0694538672240166, 0.0745521293290646, 0.0810249429717761, 0.0896658903484879, 0.102039864086428; 0.0272599116374117, 0.0274508551760269, 0.0276459635536484, 0.0278453976360045, 0.0280493324330715, 0.0282579503033167, 0.0284714477723067, 0.0286900351871743, 0.0289139377380984, 0.0291433969051845, 0.0293786719292363, 0.0296200413251744, 0.0298678048025279, 0.0301222852022004, 0.0303838306790515, 0.0306528171253096, 0.0309296508716726, 0.0312147717101397, 0.0315086562908485, 0.0318118219546270, 0.0321248310734952, 0.0324482959830040, 0.0327828835407830, 0.0331293254401937, 0.0334884201246903, 0.0338610445770192, 0.0342481649463145, 0.0346508411981931, 0.0350702483370415, 0.0355076856068923, 0.0359645941885180, 0.0364425760641698, 0.0369434156080971, 0.0374691043445147, 0.0380218694322222, 0.0386042066006265, 0.0392189184942810, 0.0398691597080478, 0.0405584902482432, 0.0412909397871346, 0.0420710859615658, 0.0429041512084280, 0.0437961243908786, 0.0447539159969595, 0.0457855593793101, 0.0469004759935903, 0.0481098309458422, 0.0494270177195512, 0.0508683346682754, 0.0524539377062183, 0.0542092314999348, 0.0561669290043804, 0.0583702038567300, 0.0608776729245815, 0.0637715776131922, 0.0671718566114411, 0.0712617378220362, 0.0763376573021695, 0.0829159379945266, 0.0919915103988414; 0.0313161453316312, 0.0315056934527626, 0.0316990547202061, 0.0318963628881813, 0.0320977597871926, 0.0323033960355761, 0.0325134317052312, 0.0327280373924446, 0.0329473949366424, 0.0331716985335869, 0.0334011558447541, 0.0336359892289973, 0.0338764371054532, 0.0341227554615844, 0.0343752195297697, 0.0346341256588640, 0.0348997934130787, 0.0351725679371764, 0.0354528226346101, 0.0357409622140073, ...(+25533 chars)] W/(m*K)  Pr_liq=[10.4273759697398, 10.4273333435620, 10.4272850929727, 10.4272304759595, 10.4271686526003, 10.4270986722631, 10.4270194589027, 10.4269297946085, 10.4268283008746, 10.4267134174688, 10.4265833785043, 10.4264361853772, 10.4262695760504, 10.4260809905276, 10.4258675315797, 10.4256259204502, 10.4253524465634, 10.4250429111609, 10.4246925633157, 10.4242960268844, 10.4238472190721, 10.4233392579372, 10.4227643578269, 10.4221137113993, 10.4213773563421, 10.4205440250291, 10.4196009748778, 10.4185337970349, 10.4173262008332, 10.4159597709726, 10.4144136941477, 10.4126644862706, 10.4106855291426, 10.4084468378503, 10.4059145337046, 10.4030503783318, 10.3998112293117, 10.3961484324846, 10.3920071452895, 10.3873255845177, 10.3820341926943, 10.3760547172142, 10.3692991965888, 10.3616688495536, 10.3530528639938, 10.3433270848464, 10.3323526031350, 10.3199742527876, 10.3060190273103, 10.2902944362434, 10.2725868312992, 10.2526597450285, 10.2302523006311, 10.2050777726083, 10.1768224028941, 10.1451446375528, 10.1096747859814, 10.0700157199265, 10.0257443762187, 9.97641472605149; 9.87159699476625, 9.83799103867815, 9.80396350066401, 9.76950431797879, 9.73460308993717, 9.69924904968617, 9.66343105461907, 9.62713751504140, 9.59035639929241, 9.55307518160880, 9.51528080644287, 9.47695964842512, 9.43809746906146, 9.39867937023294, 9.35868974438879, 9.31811222080003, 9.27692960770394, 9.23512382990164, 9.19267586114722, 9.14956565129747, 9.10577204665812, 9.06127270350925, 9.01604399697232, 8.97006091349777, 8.92329694463996, 8.87572396261244, 8.82731208731935, 8.77802954032811, 8.72784248453906, 8.67671484818998, 8.62460813144293, 8.57148119355552, 8.51729001849718, 8.46198745657646, 8.40552293933678, 8.34784216433714, 8.28888674634535, 8.22859387396988, 8.16689571152875, 8.10371915665949, 8.03898515112318, 7.97260807565909, 7.90449523035702, 7.83454568855933, 7.76264975575240, 7.68868767532505, 7.61252838493419, 7.53402791615708, 7.45302738374418, 7.36935037680814, 7.28279946463606, 7.19315135692932, 7.10014996416845, 7.00349608950524, 6.90283154977323, 6.79771372729567, 6.68757275321053, 6.57163403914766, 6.44875888619255, 6.31703791283571; 9.36056684229849, 9.29888175981754, 9.23673990094370, 9.17413356297500, 9.11105489715705, 9.04749588390381, 8.98344834420398, 8.91890384244545, 8.85385373015796, 8.78828908964791, 8.72220071106628, 8.65557906563933, 8.58841427691853, 8.52069609138865, 8.45241384790671, 8.38355644584748, 8.31411231197592, 8.24406936564880, 8.17341498236022, 8.10213595521332, 8.03021845419963, 7.95764798276762, 7.88440933340439, 7.81048652856738, 7.73586278575573, 7.66052044089047, 7.58444089466718, 7.50760454194713, 7.42999069664858, 7.35157750914387, 7.27234187534198, 7.19225933611947, 7.11130396586024, 7.02944824837767, 6.94666293826364, 6.86291690543232, 6.77817695980570, 6.69240765248036, 6.60557104880914, 6.51762646716709, 6.42853017552786, 6.33823503501912, 6.24669007595047, 6.15383992629480, 6.05962439289379, 5.96397739965884, 5.86682615395107, 5.76808980735180, 5.66767772152926, 5.56548710313451, 5.46139969930506, 5.35527706273480, 5.24695360681226, 5.13622608978612, 5.02283732379782, 4.90644994532549, 4.78660231837108, 4.66262879717945, 4.53349509512539, 4.39737461393742; 8.88957890604763, 8.80442087190143, 8.71903926749720, 8.63343144628115, 8.54759480285340, 8.46152674802285, 8.37522473389327, 8.28868613350753, 8.20190831229850, 8.11488856567849, 8.02762410329464, 7.94011202960484, 7.85234932363138, 7.76433281943496, 7.67605918697973, 7.58752491319672, 7.49872628340888, 7.40965936280273, 7.32031997801217, 7.23070371594663, 7.14080581765644, 7.05062133331172, 6.96014492748144, 6.86937094495920, 6.77829337172411, 6.68690580391799, 6.59520143334030, 6.50317300499644, 6.41081278998730, 6.31811254672793, 6.22506347848429, 6.13165618500885, 6.03788060717056, 5.94372596324150, 5.84918067522744, 5.75423228321893, 5.65886734518442, 5.56307131910738, 5.46682842315471, 5.37012146854744, 5.27293165784061, 5.17523833895514, ...(+23178 chars)]  Pr_vap=[1.00947920803444, 1.01004291823486, 1.01065965511500, 1.01133431518933, 1.01207225858964, 1.01287933352939, 1.01376190999483, 1.01472692701115, 1.01578195251918, 1.01693526110153, 1.01819592943686, 1.01957395085564, 1.02108036885805, 1.02272742812795, 1.02452900258125, 1.02649978536547, 1.02865686090750, 1.03101899176946, 1.03360697872040, 1.03644377694819, 1.03955456277267, 1.04296673419301, 1.04670982894367, 1.05081534566286, 1.05531645768164, 1.06024761514550, 1.06564403990245, 1.07154112887494, 1.07797379529992, 1.08497579281042, 1.09257908408731, 1.10081333266807, 1.10970561215315, 1.11928044003036, 1.12956025219250, 1.14056643771663, 1.15232105088355, 1.16484930883630, 1.17818296998284, 1.19236467297668, 1.20745330321237, 1.22353044907494, 1.24070802147592, 1.25913715087038, 1.27901857285843, 1.30061490792725, 1.32426555908134, 1.35040535713888, 1.37958852192126, 1.41252012785235, 1.45009863690801, 1.49347603473551, 1.54414748087562, 1.60409157423628, 1.67600020265199, 1.76367852502157, 1.87280526924811, 2.01256545162922, 2.19974597575875, 2.47118749200583; 0.974017302519303, 0.974130084887254, 0.974272434969388, 0.974445927968902, 0.974652243025218, 0.974893175609481, 0.975170652819293, 0.975486749772561, 0.975843711362895, 0.976243976279273, 0.976690205926731, 0.977185318401657, 0.977732528351675, 0.978335393648705, 0.978997869883244, 0.979724373814870, 0.980519857036854, 0.981389891243182, 0.982340834208567, 0.983379692446145, 0.984514602866890, 0.985754760320752, 0.987110638976493, 0.988594184405487, 0.990219031069311, 0.992000747838597, 0.993957114387587, 0.996108431574606, 0.998477869267403, 1.00109185555110, 1.00398051194210, 1.00717814023426, 1.01072376808799, 1.01466176266761, 1.01904252485638, 1.02392328125524, 1.02936899786208, 1.03545344877158, 1.04226048642273, 1.04988557818404, 1.05843769912884, 1.06804165312401, 1.07884120782440, 1.09100285818339, 1.10472096350656, 1.12022440442852, 1.13778543012482, 1.15773150522580, 1.18046135781185, 1.20646702834163, 1.23636469063568, 1.27093872284157, 1.31120588691674, 1.35851288661259, 1.41468905128852, 1.48229932727737, 1.56509333387213, 1.66888374269083, 1.80351410549683, 1.98818838895513; 0.961965219432596, 0.961845813603614, 0.961737514916263, 0.961641280414988, 0.961558141470659, 0.961489231891144, 0.961435785004952, 0.961399149838161, 0.961380806373283, 0.961382382416995, 0.961405673508537, 0.961452666360646, 0.961525565399957, 0.961626824132140, 0.961759181482836, 0.961925704006289, 0.962129834870944, 0.962375450657751, 0.962666927149653, 0.963009215451463, 0.963407929961538, 0.963869449923629, 0.964401067771097, 0.965011009034855, 0.965708748200551, 0.966505086854149, 0.967412373648204, 0.968444770652201, 0.969618482975056, 0.970952094308699, 0.972466918556319, 0.974187410784064, 0.976141640594391, 0.978361838462870, 0.980885027915689, 0.983753759467636, 0.987016966254130, 0.990730966651265, 0.994960646425425, 0.999780862867023, 1.00527812706919, 1.01155263965252, 1.01872078223737, 1.02691820548206, 1.03630371012192, 1.04706419866120, 1.05942109512382, 1.07363882483517, 1.09003609240857, 1.10900156891110, 1.13101541482707, 1.15668035017727, 1.18676723697617, 1.22228374060845, 1.26458272925954, 1.31553966102043, 1.37786150314316, 1.45566812912511, 1.55571545661195, 1.69042655912958; 0.954114398589080, 0.953925582411566, 0.953740551890255, 0.953559890010611, 0.953384242551335, 0.953214325460286, 0.953050933467889, 0.952894949334192, 0.952747355243732, 0.952609245298088, 0.952481840071432, 0.952366503335487, 0.952264761314433, 0.952178324883879, 0.952109115182643, 0.952059293183872, 0.952031293858027, 0.952027865660425, 0.952052116192452, 0.952107565020866, 0.952198204797544, 0.952328572006613, 0.952503828882604, 0.952729858297991, 0.953013385231875, 0.953362062118064, 0.953784675381811, 0.954291280597757, 0.954893410550092, 0.955604307187909, 0.956439191642855, 0.957415578943246, 0.958553645346606, 0.959876657802879, 0.961411477037002, 0.963189148231599, ...(+24343 chars)]  u_sat_liq=[191.795842042090; 202.020746473119; 212.428080712099; 223.023335775367; 233.812220332721; 244.800674878004; 255.994880324976; 267.401286338438; 279.026616066138; 290.877889220163; 302.962440399984; 315.287939224492; 327.862412003452; 340.694264849969; 353.792308430119; 367.165784487002; 380.824394282991; 394.778329175575; 409.038303513416; 423.615590103786; 438.522058522043; 453.770216576420; 469.373255285182; 485.345097780678; 501.700452611901; 518.454871997767; 535.624815664884; 553.227721013969; 571.282080478515; 589.807527092977; 608.824929468154; 628.356497593668; 648.425901159235; 669.058402425442; 690.281006095183; 712.122629169598; 734.614294447592; 757.789352196893; 781.683735649700; 806.336257453747; 831.788956169500; 858.087504540833; 885.281694862511; 913.426021750957; 942.580389647395; 972.810982465848; 1004.19134755560; 1036.80376816926; 1070.74103216543; 1106.10875689442; 1143.02851354854; 1181.64213083874; 1222.11778823368; 1264.65891037604; 1309.51760220335; 1357.01575949997; 1407.57990673855; 1461.80288739741; 1520.56703176343; 1585.34612557771] kJ/kg  u_sat_vap=[2437.15737300173; 2440.41264779548; 2443.71529685770; 2447.06584368792; 2450.46476476171; 2453.91248158690; 2457.40934967757; 2460.95565220151; 2464.55158455347; 2468.19724280059; 2471.89260855297; 2475.63753208786; 2479.43171341702; 2483.27468101088; 2487.16576798758; 2491.10408554180; 2495.08849339254; 2499.11756702971; 2503.18956153736; 2507.30237176801; 2511.45348862991; 2515.63995122567; 2519.85829453698; 2524.10449228142; 2528.37389446054; 2532.66115896748; 2536.96017641210; 2541.26398704414; 2545.56468829540; 2549.85333101309; 2554.11980190485; 2558.35268905488; 2562.53912658799; 2566.66461364432; 2570.71280176290; 2574.66524353094; 2578.50109389130; 2582.19675373905; 2585.72544326201; 2589.05668970973; 2592.15571063611; 2594.98266874222; 2597.49176760931; 2599.63014787883; 2601.33652937197; 2602.53952436294; 2603.15551834743; 2603.08597339853; 2602.21394769562; 2600.39952727662; 2597.47370638338; 2593.22999204088; 2587.41258169106; 2579.69923696393; 2569.67566036325; 2556.79562461244; 2540.31576778557; 2519.18177729676; 2491.81119411749; 2455.62165584668] kJ/kg  p_crit=inf MPa  critical_region=foundation.enum.critical_region.no_clip  p_crit_fraction=0.12  p_atm=0.101325 MPa  q_rev=0.01 Pa
      settings: SourceProductName=Simscape  SourceProductBaseCode=SS  InternalSimscapePortConfiguration="{\"Bottom\":[],\"Left\":[],\"Right\":[{\"id\":\"A\",\"label\":\"\",\"type\":\"foundation.two_phase_fluid.two_phase_fluid\"}],\"Top\":[]}"
  VaporMassFraction_2P : Subsystem  Description=Simscape Probe  InitFcn=|
      | unit=get_param([gcb '/PS-S'],'Unit');                                              
      | set_param(gcb, 'AttributesFormatString', '[-]');
      mask help: Simscape Probe
      settings: AttributesFormatString=[-]
      settings: CopyFcn=|
      | set_param(gcb,'LinkStatus','inactive');
      | set_param(gcb,'LinkStatus','none');
      | set_param([gcb '/Goto'],'GotoTag', [get(gcbh,'name')]);
      | set_param([gcb '/From'],'GotoTag', [get(gcbh,'name')]);
      | h = get_param([gcb, '/PS-S'], 'PortHandles');
      | set(h.Outport(1), 'SignalNameFromLabel', [get(gcbh,'name')])
      | clear h;
      settings: NameChangeFcn=|
      | set_param([gcb '/Goto'],'GotoTag', [get(gcbh,'name')]);
      | set_param([gcb '/From'],'GotoTag', [get(gcbh,'name')]);
      | h = get_param([gcb, '/PS-S'], 'PortHandles');
      | set(h.Outport(1), 'SignalNameFromLabel', [get(gcbh,'name')])
      | clear h;
      settings: OpenFcn=|
      | if exist('logsout', 'var')
      |   vname = get(gcbh,'name');
      |   fHandle = findall(0,'Tag',vname);
      |   if isempty(fHandle)
      |   figure('Tag',vname);
      |   end;
      |   figure(findobj('Tag',vname));
      |   plot(logsout.getElement([gcb, '/PS-S'], '-blockpath').Values)
      |   title(get(gcbh,'name'));
      |   ylabel(['VaporMassFraction (-)'] );
      | end
      mask Display: port_label('LConn', 1,'x');
  Velocity : Subsystem  Description=Simscape Probe  InitFcn=|
      | unit=get_param([gcb '/PS-S'],'Unit');                                              
      | set_param(gcb, 'AttributesFormatString', strcat('[', unit,']'));
      mask help: Simscape Probe
      settings: AttributesFormatString=[m/s]
      settings: CopyFcn=|
      | set_param(gcb,'LinkStatus','inactive');
      | set_param(gcb,'LinkStatus','none');
      | set_param([gcb '/Goto'],'GotoTag', [get(gcbh,'name')]);
      | set_param([gcb '/From'],'GotoTag', [get(gcbh,'name')]);
      | h = get_param([gcb, '/PS-S'], 'PortHandles');
      | set(h.Outport(1), 'SignalNameFromLabel', [get(gcbh,'name')])
      | clear h;
      settings: NameChangeFcn=|
      | set_param([gcb '/Goto'],'GotoTag', [get(gcbh,'name')]);
      | set_param([gcb '/From'],'GotoTag', [get(gcbh,'name')]);
      | h = get_param([gcb, '/PS-S'], 'PortHandles');
      | set(h.Outport(1), 'SignalNameFromLabel', [get(gcbh,'name')])
      | clear h;
      settings: OpenFcn=|
      | if exist('logsout', 'var')
      |   vname = get(gcbh,'name');
      |   fHandle = findall(0,'Tag',vname);
      |   if isempty(fHandle)
      |   figure('Tag',vname);
      |   end;
      |   figure(findobj('Tag',vname));
      |   plot(logsout.getElement([gcb, '/PS-S'], '-blockpath').Values)
      |   title(get(gcbh,'name'));
      |   ylabel(['Velocity (' get_param([gcb '/PS-S'],'Unit') ')'] );
      | end
      mask Display: port_label('LConn', 1,'V');
  Voltage : Subsystem  Description=Simscape Probe  InitFcn=|
      | unit=get_param([gcb '/PS-S'],'Unit');                                              
      | set_param(gcb, 'AttributesFormatString', strcat('[', unit,']'));
      mask help: Simscape Probe
      settings: AttributesFormatString=[V]
      settings: CopyFcn=|
      | set_param(gcb,'LinkStatus','inactive');
      | set_param(gcb,'LinkStatus','none');
      | set_param([gcb '/Goto'],'GotoTag', [get(gcbh,'name')]);
      | set_param([gcb '/From'],'GotoTag', [get(gcbh,'name')]);
      | h = get_param([gcb, '/PS-S'], 'PortHandles');
      | set(h.Outport(1), 'SignalNameFromLabel', [get(gcbh,'name')])
      | clear h;
      settings: NameChangeFcn=|
      | set_param([gcb '/Goto'],'GotoTag', [get(gcbh,'name')]);
      | set_param([gcb '/From'],'GotoTag', [get(gcbh,'name')]);
      | h = get_param([gcb, '/PS-S'], 'PortHandles');
      | set(h.Outport(1), 'SignalNameFromLabel', [get(gcbh,'name')])
      | clear h;
      settings: OpenFcn=|
      | if exist('logsout', 'var')
      |   vname = get(gcbh,'name');
      |   fHandle = findall(0,'Tag',vname);
      |   if isempty(fHandle)
      |   figure('Tag',vname);
      |   end;
      |   figure(findobj('Tag',vname));
      |   plot(logsout.getElement([gcb, '/PS-S'], '-blockpath').Values)
      |   title(get(gcbh,'name'));
      |   ylabel(['Voltage (' get_param([gcb '/PS-S'],'Unit') ')'] );
      | end
      mask Display: port_label('LConn', 1,'V');
  VolumetricFlow_2P : Subsystem  Description=Simscape Probe  InitFcn=|
      | unit=get_param([gcb '/PS-S'],'Unit');                                              
      | set_param(gcb, 'AttributesFormatString', strcat('[', unit,']'));
      mask help: Simscape Probe
      settings: AttributesFormatString=[m^3/s]
      settings: CopyFcn=|
      | if strcmp(get_param(gcb, 'LinkStatus'),'implicit') == 0;
      | set_param(gcb,'LinkStatus','inactive');
      | set_param(gcb,'LinkStatus','none');
      | end
      | set_param([gcb '/Goto'],'GotoTag', [get(gcbh,'name')]);
      | set_param([gcb '/From'],'GotoTag', [get(gcbh,'name')]);
      | h = get_param([gcb, '/PS-S'], 'PortHandles');
      | set(h.Outport(1), 'SignalNameFromLabel', [get(gcbh,'name')])
      | clear h;
      settings: NameChangeFcn=|
      | set_param([gcb '/Goto'],'GotoTag', [get(gcbh,'name')]);
      | set_param([gcb '/From'],'GotoTag', [get(gcbh,'name')]);
      | h = get_param([gcb, '/PS-S'], 'PortHandles');
      | set(h.Outport(1), 'SignalNameFromLabel', [get(gcbh,'name')])
      | clear h;
      settings: OpenFcn=|
      | if exist('logsout', 'var')
      |   vname = get(gcbh,'name');
      |   fHandle = findall(0,'Tag',vname);
      |   if isempty(fHandle)
      |   figure('Tag',vname);
      |   end;
      |   figure(findobj('Tag',vname));
      |   plot(logsout.getElement([gcb, '/PS-S'], '-blockpath').Values)
      |   title(get(gcbh,'name'));
      |   ylabel(['Volumetric Flow (' get_param([gcb '/PS-S'],'Unit') ')'] );
      | end
      mask Display:
      | patch([0.5 1 0.5], [0.25 .5 0.75],[0.7 0.7 0.7])
      | plot([0,0.5],[0.5,0.5]);
  dAngVel : Subsystem  Description=Simscape Probe  InitFcn=|
      | unit=get_param([gcb '/PS-S'],'Unit');                                              
      | set_param(gcb, 'AttributesFormatString', strcat('[', unit,']'));
      mask help: Simscape Probe
      settings: AttributesFormatString=[rad/s]
      settings: CopyFcn=|
      | set_param(gcb,'LinkStatus','inactive');
      | set_param(gcb,'LinkStatus','none');
      | set_param([gcb '/Goto'],'GotoTag', [get(gcbh,'name')]);
      | set_param([gcb '/From'],'GotoTag', [get(gcbh,'name')]);
      | h = get_param([gcb, '/PS-S'], 'PortHandles');
      | set(h.Outport(1), 'SignalNameFromLabel', [get(gcbh,'name')])
      | clear h;
      settings: NameChangeFcn=|
      | set_param([gcb '/Goto'],'GotoTag', [get(gcbh,'name')]);
      | set_param([gcb '/From'],'GotoTag', [get(gcbh,'name')]);
      | h = get_param([gcb, '/PS-S'], 'PortHandles');
      | set(h.Outport(1), 'SignalNameFromLabel', [get(gcbh,'name')])
      | clear h;
      settings: OpenFcn=|
      | if exist('logsout', 'var')
      |   vname = get(gcbh,'name');
      |   fHandle = findall(0,'Tag',vname);
      |   if isempty(fHandle)
      |   figure('Tag',vname);
      |   end;
      |   figure(findobj('Tag',vname));
      |   plot(logsout.getElement([gcb, '/PS-S'], '-blockpath').Values)
      |   title(get(gcbh,'name'));
      |   ylabel(['Angular Velocity (' get_param([gcb '/PS-S'],'Unit') ')'] );
      | end
      mask Display:
      | port_label('RConn', 1,'-');
      | port_label('LConn', 1,'+');
  dAngle : Subsystem  Description=Simscape Probe  InitFcn=|
      | unit=get_param([gcb '/PS-S'],'Unit');                                              
      | set_param(gcb, 'AttributesFormatString', strcat('[', unit,']'));
      mask help: Simscape Probe
      settings: AttributesFormatString=[rad]
      settings: CopyFcn=|
      | set_param(gcb,'LinkStatus','inactive');
      | set_param(gcb,'LinkStatus','none');
      | set_param([gcb '/Goto'],'GotoTag', [get(gcbh,'name')]);
      | set_param([gcb '/From'],'GotoTag', [get(gcbh,'name')]);
      | h = get_param([gcb, '/PS-S'], 'PortHandles');
      | set(h.Outport(1), 'SignalNameFromLabel', [get(gcbh,'name')])
      | clear h;
      settings: NameChangeFcn=|
      | set_param([gcb '/Goto'],'GotoTag', [get(gcbh,'name')]);
      | set_param([gcb '/From'],'GotoTag', [get(gcbh,'name')]);
      | h = get_param([gcb, '/PS-S'], 'PortHandles');
      | set(h.Outport(1), 'SignalNameFromLabel', [get(gcbh,'name')])
      | clear h;
      settings: OpenFcn=|
      | if exist('logsout', 'var')
      |   vname = get(gcbh,'name');
      |   fHandle = findall(0,'Tag',vname);
      |   if isempty(fHandle)
      |   figure('Tag',vname);
      |   end;
      |   figure(findobj('Tag',vname));
      |   plot(logsout.getElement([gcb, '/PS-S'], '-blockpath').Values)
      |   title(get(gcbh,'name'));
      |   ylabel(['Angle (' get_param([gcb '/PS-S'],'Unit') ')'] );
      | end
      mask Display:
      | port_label('RConn', 1,'-');
      | port_label('LConn', 1,'+');
  dEnergy_2P : Subsystem  Description=Simscape Probe  InitFcn=|
      | unit=get_param([gcb '/PS-S'],'Unit');                                              
      | set_param(gcb, 'AttributesFormatString', strcat('[', unit,']'));
      mask help: Simscape Probe
      settings: AttributesFormatString=[kJ/kg]
      settings: CopyFcn=|
      | if strcmp(get_param(gcb, 'LinkStatus'),'implicit') == 0;
      | set_param(gcb,'LinkStatus','inactive');
      | set_param(gcb,'LinkStatus','none');
      | end
      | set_param([gcb '/Goto'],'GotoTag', [get(gcbh,'name')]);
      | set_param([gcb '/From'],'GotoTag', [get(gcbh,'name')]);
      | h = get_param([gcb, '/PS-S'], 'PortHandles');
      | set(h.Outport(1), 'SignalNameFromLabel', [get(gcbh,'name')])
      | clear h;
      settings: NameChangeFcn=|
      | set_param([gcb '/Goto'],'GotoTag', [get(gcbh,'name')]);
      | set_param([gcb '/From'],'GotoTag', [get(gcbh,'name')]);
      | h = get_param([gcb, '/PS-S'], 'PortHandles');
      | set(h.Outport(1), 'SignalNameFromLabel', [get(gcbh,'name')])
      | clear h;
      settings: OpenFcn=|
      | if exist('logsout', 'var')
      |   vname = get(gcbh,'name');
      |   fHandle = findall(0,'Tag',vname);
      |   if isempty(fHandle)
      |   figure('Tag',vname);
      |   end;
      |   figure(findobj('Tag',vname));
      |   plot(logsout.getElement([gcb, '/PS-S'], '-blockpath').Values)
      |   title(get(gcbh,'name'));
      |   ylabel(['Temperature (' get_param([gcb '/PS-S'],'Unit') ')'] );
      | end
      mask Display:
      | port_label('RConn', 1,'-');
      | port_label('LConn', 1,'+');
  dGasPressure : Subsystem  Description=Simscape Probe  InitFcn=|
      | unit=get_param([gcb '/PS-S'],'Unit');                                              
      | set_param(gcb, 'AttributesFormatString', strcat('[', unit,']'));
      mask help: Simscape Probe
      settings: AttributesFormatString=[Pa]
      settings: CopyFcn=|
      | set_param(gcb,'LinkStatus','inactive');
      | set_param(gcb,'LinkStatus','none');
      | set_param([gcb '/Goto'],'GotoTag', [get(gcbh,'name')]);
      | set_param([gcb '/From'],'GotoTag', [get(gcbh,'name')]);
      | h = get_param([gcb, '/PS-S'], 'PortHandles');
      | set(h.Outport(1), 'SignalNameFromLabel', [get(gcbh,'name')])
      | clear h;
      settings: NameChangeFcn=|
      | set_param([gcb '/Goto'],'GotoTag', [get(gcbh,'name')]);
      | set_param([gcb '/From'],'GotoTag', [get(gcbh,'name')]);
      | h = get_param([gcb, '/PS-S'], 'PortHandles');
      | set(h.Outport(1), 'SignalNameFromLabel', [get(gcbh,'name')])
      | clear h;
      settings: OpenFcn=|
      | if exist('logsout', 'var')
      |   vname = get(gcbh,'name');
      |   fHandle = findall(0,'Tag',vname);
      |   if isempty(fHandle)
      |   figure('Tag',vname);
      |   end;
      |   figure(findobj('Tag',vname));
      |   plot(logsout.getElement([gcb, '/PS-S'], '-blockpath').Values)
      |   title(get(gcbh,'name'));
      |   ylabel(['Pressure (' get_param([gcb '/PS-S'],'Unit') ')'] );
      | end
      mask Display:
      | port_label('RConn', 1,'-');
      | port_label('LConn', 1,'+');
  dGasTemperature : Subsystem  Description=Simscape Probe  InitFcn=|
      | unit=get_param([gcb '/PS-S'],'Unit');                                              
      | set_param(gcb, 'AttributesFormatString', strcat('[', unit,']'));
      mask help: Simscape Probe
      settings: AttributesFormatString=[K]
      settings: CopyFcn=|
      | set_param(gcb,'LinkStatus','inactive');
      | set_param(gcb,'LinkStatus','none');
      | set_param([gcb '/Goto'],'GotoTag', [get(gcbh,'name')]);
      | set_param([gcb '/From'],'GotoTag', [get(gcbh,'name')]);
      | h = get_param([gcb, '/PS-S'], 'PortHandles');
      | set(h.Outport(1), 'SignalNameFromLabel', [get(gcbh,'name')])
      | clear h;
      settings: NameChangeFcn=|
      | set_param([gcb '/Goto'],'GotoTag', [get(gcbh,'name')]);
      | set_param([gcb '/From'],'GotoTag', [get(gcbh,'name')]);
      | h = get_param([gcb, '/PS-S'], 'PortHandles');
      | set(h.Outport(1), 'SignalNameFromLabel', [get(gcbh,'name')])
      | clear h;
      settings: OpenFcn=|
      | if exist('logsout', 'var')
      |   vname = get(gcbh,'name');
      |   fHandle = findall(0,'Tag',vname);
      |   if isempty(fHandle)
      |   figure('Tag',vname);
      |   end;
      |   figure(findobj('Tag',vname));
      |   plot(logsout.getElement([gcb, '/PS-S'], '-blockpath').Values)
      |   title(get(gcbh,'name'));
      |   ylabel(['Temperature (' get_param([gcb '/PS-S'],'Unit') ')'] );
      | end
      mask Display:
      | port_label('RConn', 1,'-');
      | port_label('LConn', 1,'+');
  dMMF : Subsystem  Description=Simscape Probe  InitFcn=|
      | unit=get_param([gcb '/PS-S'],'Unit');                                              
      | set_param(gcb, 'AttributesFormatString', strcat('[', unit,']'));
      mask help: Simscape Probe
      settings: AttributesFormatString=[A]
      settings: CopyFcn=|
      | set_param(gcb,'LinkStatus','inactive');
      | set_param(gcb,'LinkStatus','none');
      | set_param([gcb '/Goto'],'GotoTag', [get(gcbh,'name')]);
      | set_param([gcb '/From'],'GotoTag', [get(gcbh,'name')]);
      | h = get_param([gcb, '/PS-S'], 'PortHandles');
      | set(h.Outport(1), 'SignalNameFromLabel', [get(gcbh,'name')])
      | clear h;
      settings: NameChangeFcn=|
      | set_param([gcb '/Goto'],'GotoTag', [get(gcbh,'name')]);
      | set_param([gcb '/From'],'GotoTag', [get(gcbh,'name')]);
      | h = get_param([gcb, '/PS-S'], 'PortHandles');
      | set(h.Outport(1), 'SignalNameFromLabel', [get(gcbh,'name')])
      | clear h;
      settings: OpenFcn=|
      | if exist('logsout', 'var')
      |   vname = get(gcbh,'name');
      |   fHandle = findall(0,'Tag',vname);
      |   if isempty(fHandle)
      |   figure('Tag',vname);
      |   end;
      |   figure(findobj('Tag',vname));
      |   plot(logsout.getElement([gcb, '/PS-S'], '-blockpath').Values)
      |   title(get(gcbh,'name'));
      |   ylabel(['MMF (' get_param([gcb '/PS-S'],'Unit') ')'] );
      | end
      mask Display:
      | port_label('RConn', 1,'-');
      | port_label('LConn', 1,'+');
  dPosition : Subsystem  Description=Simscape Probe  InitFcn=|
      | unit=get_param([gcb '/PS-S'],'Unit');                                              
      | set_param(gcb, 'AttributesFormatString', strcat('[', unit,']'));
      mask help: Simscape Probe
      settings: AttributesFormatString=[m]
      settings: CopyFcn=|
      | set_param(gcb,'LinkStatus','inactive');
      | set_param(gcb,'LinkStatus','none');
      | set_param([gcb '/Goto'],'GotoTag', [get(gcbh,'name')]);
      | set_param([gcb '/From'],'GotoTag', [get(gcbh,'name')]);
      | h = get_param([gcb, '/PS-S'], 'PortHandles');
      | set(h.Outport(1), 'SignalNameFromLabel', [get(gcbh,'name')])
      | clear h;
      settings: NameChangeFcn=|
      | set_param([gcb '/Goto'],'GotoTag', [get(gcbh,'name')]);
      | set_param([gcb '/From'],'GotoTag', [get(gcbh,'name')]);
      | h = get_param([gcb, '/PS-S'], 'PortHandles');
      | set(h.Outport(1), 'SignalNameFromLabel', [get(gcbh,'name')])
      | clear h;
      settings: OpenFcn=|
      | if exist('logsout', 'var')
      |   vname = get(gcbh,'name');
      |   fHandle = findall(0,'Tag',vname);
      |   if isempty(fHandle)
      |   figure('Tag',vname);
      |   end;
      |   figure(findobj('Tag',vname));
      |   plot(logsout.getElement([gcb, '/PS-S'], '-blockpath').Values)
      |   title(get(gcbh,'name'));
      |   ylabel(['Position (' get_param([gcb '/PS-S'],'Unit') ')'] );
      | end
      mask Display:
      | port_label('RConn', 1,'-');
      | port_label('LConn', 1,'+');
  dPressure : Subsystem  Description=Simscape Probe  InitFcn=|
      | unit=get_param([gcb '/PS-S'],'Unit');                                             
      | set_param(gcb, 'AttributesFormatString', strcat('[', unit,']'));
      mask help: Simscape Probe
      settings: AttributesFormatString=[Pa]
      settings: CopyFcn=|
      | set_param(gcb,'LinkStatus','inactive');
      | set_param(gcb,'LinkStatus','none');
      | set_param([gcb '/Goto'],'GotoTag', [get(gcbh,'name')]);
      | set_param([gcb '/From'],'GotoTag', [get(gcbh,'name')]);
      | h = get_param([gcb, '/PS-S'], 'PortHandles');
      | set(h.Outport(1), 'SignalNameFromLabel', [get(gcbh,'name')])
      | clear h;
      settings: NameChangeFcn=|
      | set_param([gcb '/Goto'],'GotoTag', [get(gcbh,'name')]);
      | set_param([gcb '/From'],'GotoTag', [get(gcbh,'name')]);
      | h = get_param([gcb, '/PS-S'], 'PortHandles');
      | set(h.Outport(1), 'SignalNameFromLabel', [get(gcbh,'name')])
      | clear h;
      settings: OpenFcn=|
      | if exist('logsout', 'var')
      |   vname = get(gcbh,'name');
      |   fHandle = findall(0,'Tag',vname);
      |   if isempty(fHandle)
      |   figure('Tag',vname);
      |   end;
      |   figure(findobj('Tag',vname));
      |   plot(logsout.getElement([gcb, '/PS-S'], '-blockpath').Values)
      |   title(get(gcbh,'name'));
      |   ylabel(['Pressure (' get_param([gcb '/PS-S'],'Unit') ')'] );
      | end
      mask Display:
      | port_label('RConn', 1,'-');
      | port_label('LConn', 1,'+');
  dPressure_2P : Subsystem  Description=Simscape Probe  InitFcn=|
      | unit=get_param([gcb '/PS-S'],'Unit');                                              
      | set_param(gcb, 'AttributesFormatString', strcat('[', unit,']'));
      mask help: Simscape Probe
      settings: AttributesFormatString=[Pa]
      settings: CopyFcn=|
      | if strcmp(get_param(gcb, 'LinkStatus'),'implicit') == 0;
      | set_param(gcb,'LinkStatus','inactive');
      | set_param(gcb,'LinkStatus','none');
      | end
      | set_param([gcb '/Goto'],'GotoTag', [get(gcbh,'name')]);
      | set_param([gcb '/From'],'GotoTag', [get(gcbh,'name')]);
      | h = get_param([gcb, '/PS-S'], 'PortHandles');
      | set(h.Outport(1), 'SignalNameFromLabel', [get(gcbh,'name')])
      | clear h;
      settings: NameChangeFcn=|
      | set_param([gcb '/Goto'],'GotoTag', [get(gcbh,'name')]);
      | set_param([gcb '/From'],'GotoTag', [get(gcbh,'name')]);
      | h = get_param([gcb, '/PS-S'], 'PortHandles');
      | set(h.Outport(1), 'SignalNameFromLabel', [get(gcbh,'name')])
      | clear h;
      settings: OpenFcn=|
      | if exist('logsout', 'var')
      |   vname = get(gcbh,'name');
      |   fHandle = findall(0,'Tag',vname);
      |   if isempty(fHandle)
      |   figure('Tag',vname);
      |   end;
      |   figure(findobj('Tag',vname));
      |   plot(logsout.getElement([gcb, '/PS-S'], '-blockpath').Values)
      |   title(get(gcbh,'name'));
      |   ylabel(['Pressure (' get_param([gcb '/PS-S'],'Unit') ')'] );
      | end
      mask Display:
      | port_label('RConn', 1,'-');
      | port_label('LConn', 1,'+');
  dPressure_TL : Subsystem  Description=Simscape Probe  InitFcn=|
      | unit=get_param([gcb '/PS-S'],'Unit');                                              
      | set_param(gcb, 'AttributesFormatString', strcat('[', unit,']'));
      mask help: Simscape Probe
      settings: AttributesFormatString=[Pa]
      settings: CopyFcn=|
      | set_param(gcb,'LinkStatus','inactive');
      | set_param(gcb,'LinkStatus','none');
      | set_param([gcb '/Goto'],'GotoTag', [get(gcbh,'name')]);
      | set_param([gcb '/From'],'GotoTag', [get(gcbh,'name')]);
      | h = get_param([gcb, '/PS-S'], 'PortHandles');
      | set(h.Outport(1), 'SignalNameFromLabel', [get(gcbh,'name')])
      | clear h;
      settings: NameChangeFcn=|
      | set_param([gcb '/Goto'],'GotoTag', [get(gcbh,'name')]);
      | set_param([gcb '/From'],'GotoTag', [get(gcbh,'name')]);
      | h = get_param([gcb, '/PS-S'], 'PortHandles');
      | set(h.Outport(1), 'SignalNameFromLabel', [get(gcbh,'name')])
      | clear h;
      settings: OpenFcn=|
      | if exist('logsout', 'var')
      |   vname = get(gcbh,'name');
      |   fHandle = findall(0,'Tag',vname);
      |   if isempty(fHandle)
      |   figure('Tag',vname);
      |   end;
      |   figure(findobj('Tag',vname));
      |   plot(logsout.getElement([gcb, '/PS-S'], '-blockpath').Values)
      |   title(get(gcbh,'name'));
      |   ylabel(['Pressure (' get_param([gcb '/PS-S'],'Unit') ')'] );
      | end
      mask Display:
      | port_label('RConn', 1,'-');
      | port_label('LConn', 1,'+');
  dTemperature : Subsystem  Description=Simscape Probe  InitFcn=|
      | unit=get_param([gcb '/PS-S'],'Unit');                                              
